simulink model "autoCreatedModel"  (R2023a)
settings: Solver=FixedStepDiscrete  StartTime=0.0  StopTime=10.0  FixedStep=0.1  RelTol=1e-3
undefined symbols (not defined in the file or in its folder): Batt_AncOutVoltage, Batt_BalancingRequired, Batt_BMSStatus, Batt_BoostChargeActive, Batt_ChargeContactorStatus, Batt_ClearFault_Code, Batt_ClearFault_KeyMatched, Batt_Coolant_IN_Pressure, Batt_Coolant_IN_Temp, Batt_Coolant_OUT_Pressure, Batt_Coolant_OUT_Temp, Batt_Current, Batt_DischargePowerLim, Batt_DischargePowerLim_2s, Batt_DischargePowerLim_5s, Batt_DischEnergyThroughput, Batt_EnergyAvailable, Batt_Equity_SoC_Displayed, Batt_Fault_FR0, Batt_Fault_FR1, Batt_Fault_FR2, Batt_Fault_FR3, Batt_Fault_FR4, Batt_Fault_FR5, Batt_Fault_FR6, Batt_Fault_FR7, Batt_FaultActive_FR4, Batt_HVILFault, Batt_InvOutVoltage, Batt_Isolation1OnOffStatus, Batt_Isolation1Res_HighRange, Batt_Isolation1Resistance, Batt_Isolation1Status, Batt_Isolation2OnOffStatus, Batt_Isolation2Status, Batt_LoggerPercent, Batt_LVBackupBattVoltage, Batt_LVVoltage, Batt_MainContactorStatus, Batt_MaxCellTemperature, Batt_MaxCellVoltage, Batt_MaxSOC, Batt_MinCellTemperature, Batt_MinCellVoltage, Batt_MinSOC, Batt_ReadyforBoostCharge, Batt_ReadytoTurnOnHV, Batt_RegenPowerLim, Batt_RegenPowerLim_2s, Batt_RegenPowerLim_5s, Batt_SafetyLightStatGreenHV, Batt_SafetyLightStatRedHV, Batt_SerialNumber, Batt_ThermalRequest, Batt_UserSOC, Batt_Voltage, BMS, BMS_AliveCounter1, BMS_AliveCounter2, BMS_AliveCounter3 ... (+154)
libraries: canoelib x133
(part 2 of 2)

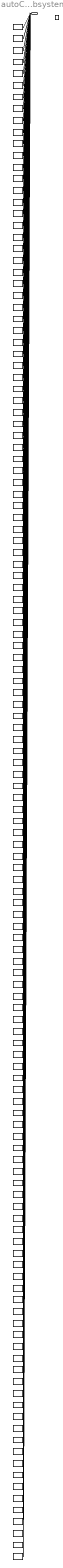
== system autoCreatedModel/BMS_EnabledSubsystem ==
  Enable : EnablePort
  En_OverRide_BMS_AliveCounter1 : canoelib/CANoe I//O/System Variable Input  nsName=HIL_Interface  sysVarName=CAN_OverRide::BMS::xC9_BMS_HV_01_Status::BMS_AliveCounter1::En_OverRide_BMS_AliveCounter1  arrayIndex=-1  editSampleTime=0.001  rawValue=Default  dataType=Default  dataTypeDB=unknown  hasEncoding=off  dataTypeCANoe=Get from CANoe
      settings: AttributesFormatString=%<nsName>::%<sysVarName>  SourceProductName=Vector CANoe
  En_OverRide_BMS_AliveCounter2 : canoelib/CANoe I//O/System Variable Input  nsName=HIL_Interface  sysVarName=CAN_OverRide::BMS::xCA_BMS_HV_02_HVParameter::BMS_AliveCounter2::En_OverRide_BMS_AliveCounter2  arrayIndex=-1  editSampleTime=0.001  rawValue=Default  dataType=Default  dataTypeDB=unknown  hasEncoding=off  dataTypeCANoe=Get from CANoe
      settings: AttributesFormatString=%<nsName>::%<sysVarName>  SourceProductName=Vector CANoe
  En_OverRide_BMS_AliveCounter3 : canoelib/CANoe I//O/System Variable Input  nsName=HIL_Interface  sysVarName=CAN_OverRide::BMS::xCB_BMS_HV_03_BatteryLimits::BMS_AliveCounter3::En_OverRide_BMS_AliveCounter3  arrayIndex=-1  editSampleTime=0.001  rawValue=Default  dataType=Default  dataTypeDB=unknown  hasEncoding=off  dataTypeCANoe=Get from CANoe
      settings: AttributesFormatString=%<nsName>::%<sysVarName>  SourceProductName=Vector CANoe
  En_OverRide_BMS_Calibration_info : canoelib/CANoe I//O/System Variable Input  nsName=HIL_Interface  sysVarName=CAN_OverRide::BMS::x112_BMS_HV_12::BMS_Calibration_info::En_OverRide_BMS_Calibration_info  arrayIndex=-1  editSampleTime=0.001  rawValue=Default  dataType=Default  dataTypeDB=unknown  hasEncoding=off  dataTypeCANoe=Get from CANoe
      settings: AttributesFormatString=%<nsName>::%<sysVarName>  SourceProductName=Vector CANoe
  En_OverRide_BMS_LoggingFull : canoelib/CANoe I//O/System Variable Input  nsName=HIL_Interface  sysVarName=CAN_OverRide::BMS::x110_BMS_HV_09::BMS_LoggingFull::En_OverRide_BMS_LoggingFull  arrayIndex=-1  editSampleTime=0.001  rawValue=Default  dataType=Default  dataTypeDB=unknown  hasEncoding=off  dataTypeCANoe=Get from CANoe
      settings: AttributesFormatString=%<nsName>::%<sysVarName>  SourceProductName=Vector CANoe
  En_OverRide_BMS_Software_info : canoelib/CANoe I//O/System Variable Input  nsName=HIL_Interface  sysVarName=CAN_OverRide::BMS::x112_BMS_HV_12::BMS_Software_info::En_OverRide_BMS_Software_info  arrayIndex=-1  editSampleTime=0.001  rawValue=Default  dataType=Default  dataTypeDB=unknown  hasEncoding=off  dataTypeCANoe=Get from CANoe
      settings: AttributesFormatString=%<nsName>::%<sysVarName>  SourceProductName=Vector CANoe
  En_OverRide_Batt_AncOutVoltage : canoelib/CANoe I//O/System Variable Input  nsName=HIL_Interface  sysVarName=CAN_OverRide::BMS::xCC_BMS_HV_04_ContactorStatus::Batt_AncOutVoltage::En_OverRide_Batt_AncOutVoltage  arrayIndex=-1  editSampleTime=0.001  rawValue=Default  dataType=Default  dataTypeDB=unknown  hasEncoding=off  dataTypeCANoe=Get from CANoe
      settings: AttributesFormatString=%<nsName>::%<sysVarName>  SourceProductName=Vector CANoe
  En_OverRide_Batt_BMSStatus : canoelib/CANoe I//O/System Variable Input  nsName=HIL_Interface  sysVarName=CAN_OverRide::BMS::xC9_BMS_HV_01_Status::Batt_BMSStatus::En_OverRide_Batt_BMSStatus  arrayIndex=-1  editSampleTime=0.001  rawValue=Default  dataType=Default  dataTypeDB=unknown  hasEncoding=off  dataTypeCANoe=Get from CANoe
      settings: AttributesFormatString=%<nsName>::%<sysVarName>  SourceProductName=Vector CANoe
  En_OverRide_Batt_BalancingRequired : canoelib/CANoe I//O/System Variable Input  nsName=HIL_Interface  sysVarName=CAN_OverRide::BMS::xC9_BMS_HV_01_Status::Batt_BalancingRequired::En_OverRide_Batt_BalancingRequired  arrayIndex=-1  editSampleTime=0.001  rawValue=Default  dataType=Default  dataTypeDB=unknown  hasEncoding=off  dataTypeCANoe=Get from CANoe
      settings: AttributesFormatString=%<nsName>::%<sysVarName>  SourceProductName=Vector CANoe
  En_OverRide_Batt_BoostChargeActive : canoelib/CANoe I//O/System Variable Input  nsName=HIL_Interface  sysVarName=CAN_OverRide::BMS::xD2_BMS_HV_08::Batt_BoostChargeActive::En_OverRide_Batt_BoostChargeActive  arrayIndex=-1  editSampleTime=0.001  rawValue=Default  dataType=Default  dataTypeDB=unknown  hasEncoding=off  dataTypeCANoe=Get from CANoe
      settings: AttributesFormatString=%<nsName>::%<sysVarName>  SourceProductName=Vector CANoe
  En_OverRide_Batt_ChargeContactorStatus : canoelib/CANoe I//O/System Variable Input  nsName=HIL_Interface  sysVarName=CAN_OverRide::BMS::xCC_BMS_HV_04_ContactorStatus::Batt_ChargeContactorStatus::En_OverRide_Batt_ChargeContactorStatus  arrayIndex=-1  editSampleTime=0.001  rawValue=Default  dataType=Default  dataTypeDB=unknown  hasEncoding=off  dataTypeCANoe=Get from CANoe
      settings: AttributesFormatString=%<nsName>::%<sysVarName>  SourceProductName=Vector CANoe
  En_OverRide_Batt_ClearFault_Code : canoelib/CANoe I//O/System Variable Input  nsName=HIL_Interface  sysVarName=CAN_OverRide::BMS::x110_BMS_HV_09::Batt_ClearFault_Code::En_OverRide_Batt_ClearFault_Code  arrayIndex=-1  editSampleTime=0.001  rawValue=Default  dataType=Default  dataTypeDB=unknown  hasEncoding=off  dataTypeCANoe=Get from CANoe
      settings: AttributesFormatString=%<nsName>::%<sysVarName>  SourceProductName=Vector CANoe
  En_OverRide_Batt_ClearFault_KeyMatched : canoelib/CANoe I//O/System Variable Input  nsName=HIL_Interface  sysVarName=CAN_OverRide::BMS::x110_BMS_HV_09::Batt_ClearFault_KeyMatched::En_OverRide_Batt_ClearFault_KeyMatched  arrayIndex=-1  editSampleTime=0.001  rawValue=Default  dataType=Default  dataTypeDB=unknown  hasEncoding=off  dataTypeCANoe=Get from CANoe
      settings: AttributesFormatString=%<nsName>::%<sysVarName>  SourceProductName=Vector CANoe
  En_OverRide_Batt_Coolant_IN_Pressure : canoelib/CANoe I//O/System Variable Input  nsName=HIL_Interface  sysVarName=CAN_OverRide::BMS::xCF_BMS_HV_07_Thermal::Batt_Coolant_IN_Pressure::En_OverRide_Batt_Coolant_IN_Pressure  arrayIndex=-1  editSampleTime=0.001  rawValue=Default  dataType=Default  dataTypeDB=unknown  hasEncoding=off  dataTypeCANoe=Get from CANoe
      settings: AttributesFormatString=%<nsName>::%<sysVarName>  SourceProductName=Vector CANoe
  En_OverRide_Batt_Coolant_IN_Temp : canoelib/CANoe I//O/System Variable Input  nsName=HIL_Interface  sysVarName=CAN_OverRide::BMS::xCF_BMS_HV_07_Thermal::Batt_Coolant_IN_Temp::En_OverRide_Batt_Coolant_IN_Temp  arrayIndex=-1  editSampleTime=0.001  rawValue=Default  dataType=Default  dataTypeDB=unknown  hasEncoding=off  dataTypeCANoe=Get from CANoe
      settings: AttributesFormatString=%<nsName>::%<sysVarName>  SourceProductName=Vector CANoe
  En_OverRide_Batt_Coolant_OUT_Pressure : canoelib/CANoe I//O/System Variable Input  nsName=HIL_Interface  sysVarName=CAN_OverRide::BMS::xCF_BMS_HV_07_Thermal::Batt_Coolant_OUT_Pressure::En_OverRide_Batt_Coolant_OUT_Pressure  arrayIndex=-1  editSampleTime=0.001  rawValue=Default  dataType=Default  dataTypeDB=unknown  hasEncoding=off  dataTypeCANoe=Get from CANoe
      settings: AttributesFormatString=%<nsName>::%<sysVarName>  SourceProductName=Vector CANoe
  En_OverRide_Batt_Coolant_OUT_Temp : canoelib/CANoe I//O/System Variable Input  nsName=HIL_Interface  sysVarName=CAN_OverRide::BMS::xCF_BMS_HV_07_Thermal::Batt_Coolant_OUT_Temp::En_OverRide_Batt_Coolant_OUT_Temp  arrayIndex=-1  editSampleTime=0.001  rawValue=Default  dataType=Default  dataTypeDB=unknown  hasEncoding=off  dataTypeCANoe=Get from CANoe
      settings: AttributesFormatString=%<nsName>::%<sysVarName>  SourceProductName=Vector CANoe
  En_OverRide_Batt_Current : canoelib/CANoe I//O/System Variable Input  nsName=HIL_Interface  sysVarName=CAN_OverRide::BMS::xCA_BMS_HV_02_HVParameter::Batt_Current::En_OverRide_Batt_Current  arrayIndex=-1  editSampleTime=0.001  rawValue=Default  dataType=Default  dataTypeDB=unknown  hasEncoding=off  dataTypeCANoe=Get from CANoe
      settings: AttributesFormatString=%<nsName>::%<sysVarName>  SourceProductName=Vector CANoe
  En_OverRide_Batt_DischEnergyThroughput : canoelib/CANoe I//O/System Variable Input  nsName=HIL_Interface  sysVarName=CAN_OverRide::BMS::xD2_BMS_HV_08::Batt_DischEnergyThroughput::En_OverRide_Batt_DischEnergyThroughput  arrayIndex=-1  editSampleTime=0.001  rawValue=Default  dataType=Default  dataTypeDB=unknown  hasEncoding=off  dataTypeCANoe=Get from CANoe
      settings: AttributesFormatString=%<nsName>::%<sysVarName>  SourceProductName=Vector CANoe
  En_OverRide_Batt_DischargePowerLim : canoelib/CANoe I//O/System Variable Input  nsName=HIL_Interface  sysVarName=CAN_OverRide::BMS::xCB_BMS_HV_03_BatteryLimits::Batt_DischargePowerLim::En_OverRide_Batt_DischargePowerLim  arrayIndex=-1  editSampleTime=0.001  rawValue=Default  dataType=Default  dataTypeDB=unknown  hasEncoding=off  dataTypeCANoe=Get from CANoe
      settings: AttributesFormatString=%<nsName>::%<sysVarName>  SourceProductName=Vector CANoe
  En_OverRide_Batt_DischargePowerLim_2s : canoelib/CANoe I//O/System Variable Input  nsName=HIL_Interface  sysVarName=CAN_OverRide::BMS::x109_BMS_HV_10::Batt_DischargePowerLim_2s::En_OverRide_Batt_DischargePowerLim_2s  arrayIndex=-1  editSampleTime=0.001  rawValue=Default  dataType=Default  dataTypeDB=unknown  hasEncoding=off  dataTypeCANoe=Get from CANoe
      settings: AttributesFormatString=%<nsName>::%<sysVarName>  SourceProductName=Vector CANoe
  En_OverRide_Batt_DischargePowerLim_5s : canoelib/CANoe I//O/System Variable Input  nsName=HIL_Interface  sysVarName=CAN_OverRide::BMS::x109_BMS_HV_10::Batt_DischargePowerLim_5s::En_OverRide_Batt_DischargePowerLim_5s  arrayIndex=-1  editSampleTime=0.001  rawValue=Default  dataType=Default  dataTypeDB=unknown  hasEncoding=off  dataTypeCANoe=Get from CANoe
      settings: AttributesFormatString=%<nsName>::%<sysVarName>  SourceProductName=Vector CANoe
  En_OverRide_Batt_EnergyAvailable : canoelib/CANoe I//O/System Variable Input  nsName=HIL_Interface  sysVarName=CAN_OverRide::BMS::xCE_BMS_HV_06::Batt_EnergyAvailable::En_OverRide_Batt_EnergyAvailable  arrayIndex=-1  editSampleTime=0.001  rawValue=Default  dataType=Default  dataTypeDB=unknown  hasEncoding=off  dataTypeCANoe=Get from CANoe
      settings: AttributesFormatString=%<nsName>::%<sysVarName>  SourceProductName=Vector CANoe
  En_OverRide_Batt_Equity_SoC_Displayed : canoelib/CANoe I//O/System Variable Input  nsName=HIL_Interface  sysVarName=CAN_OverRide::BMS::xC9_BMS_HV_01_Status::Batt_Equity_SoC_Displayed::En_OverRide_Batt_Equity_SoC_Displayed  arrayIndex=-1  editSampleTime=0.001  rawValue=Default  dataType=Default  dataTypeDB=unknown  hasEncoding=off  dataTypeCANoe=Get from CANoe
      settings: AttributesFormatString=%<nsName>::%<sysVarName>  SourceProductName=Vector CANoe
  En_OverRide_Batt_FaultActive_FR4 : canoelib/CANoe I//O/System Variable Input  nsName=HIL_Interface  sysVarName=CAN_OverRide::BMS::x110_BMS_HV_09::Batt_FaultActive_FR4::En_OverRide_Batt_FaultActive_FR4  arrayIndex=-1  editSampleTime=0.001  rawValue=Default  dataType=Default  dataTypeDB=unknown  hasEncoding=off  dataTypeCANoe=Get from CANoe
      settings: AttributesFormatString=%<nsName>::%<sysVarName>  SourceProductName=Vector CANoe
  En_OverRide_Batt_Fault_FR0 : canoelib/CANoe I//O/System Variable Input  nsName=HIL_Interface  sysVarName=CAN_OverRide::BMS::xC9_BMS_HV_01_Status::Batt_Fault_FR0::En_OverRide_Batt_Fault_FR0  arrayIndex=-1  editSampleTime=0.001  rawValue=Default  dataType=Default  dataTypeDB=unknown  hasEncoding=off  dataTypeCANoe=Get from CANoe
      settings: AttributesFormatString=%<nsName>::%<sysVarName>  SourceProductName=Vector CANoe
  En_OverRide_Batt_Fault_FR1 : canoelib/CANoe I//O/System Variable Input  nsName=HIL_Interface  sysVarName=CAN_OverRide::BMS::xC9_BMS_HV_01_Status::Batt_Fault_FR1::En_OverRide_Batt_Fault_FR1  arrayIndex=-1  editSampleTime=0.001  rawValue=Default  dataType=Default  dataTypeDB=unknown  hasEncoding=off  dataTypeCANoe=Get from CANoe
      settings: AttributesFormatString=%<nsName>::%<sysVarName>  SourceProductName=Vector CANoe
  En_OverRide_Batt_Fault_FR2 : canoelib/CANoe I//O/System Variable Input  nsName=HIL_Interface  sysVarName=CAN_OverRide::BMS::xC9_BMS_HV_01_Status::Batt_Fault_FR2::En_OverRide_Batt_Fault_FR2  arrayIndex=-1  editSampleTime=0.001  rawValue=Default  dataType=Default  dataTypeDB=unknown  hasEncoding=off  dataTypeCANoe=Get from CANoe
      settings: AttributesFormatString=%<nsName>::%<sysVarName>  SourceProductName=Vector CANoe
  En_OverRide_Batt_Fault_FR3 : canoelib/CANoe I//O/System Variable Input  nsName=HIL_Interface  sysVarName=CAN_OverRide::BMS::xC9_BMS_HV_01_Status::Batt_Fault_FR3::En_OverRide_Batt_Fault_FR3  arrayIndex=-1  editSampleTime=0.001  rawValue=Default  dataType=Default  dataTypeDB=unknown  hasEncoding=off  dataTypeCANoe=Get from CANoe
      settings: AttributesFormatString=%<nsName>::%<sysVarName>  SourceProductName=Vector CANoe
  En_OverRide_Batt_Fault_FR4 : canoelib/CANoe I//O/System Variable Input  nsName=HIL_Interface  sysVarName=CAN_OverRide::BMS::xC9_BMS_HV_01_Status::Batt_Fault_FR4::En_OverRide_Batt_Fault_FR4  arrayIndex=-1  editSampleTime=0.001  rawValue=Default  dataType=Default  dataTypeDB=unknown  hasEncoding=off  dataTypeCANoe=Get from CANoe
      settings: AttributesFormatString=%<nsName>::%<sysVarName>  SourceProductName=Vector CANoe
  En_OverRide_Batt_Fault_FR5 : canoelib/CANoe I//O/System Variable Input  nsName=HIL_Interface  sysVarName=CAN_OverRide::BMS::xC9_BMS_HV_01_Status::Batt_Fault_FR5::En_OverRide_Batt_Fault_FR5  arrayIndex=-1  editSampleTime=0.001  rawValue=Default  dataType=Default  dataTypeDB=unknown  hasEncoding=off  dataTypeCANoe=Get from CANoe
      settings: AttributesFormatString=%<nsName>::%<sysVarName>  SourceProductName=Vector CANoe
  En_OverRide_Batt_Fault_FR6 : canoelib/CANoe I//O/System Variable Input  nsName=HIL_Interface  sysVarName=CAN_OverRide::BMS::xC9_BMS_HV_01_Status::Batt_Fault_FR6::En_OverRide_Batt_Fault_FR6  arrayIndex=-1  editSampleTime=0.001  rawValue=Default  dataType=Default  dataTypeDB=unknown  hasEncoding=off  dataTypeCANoe=Get from CANoe
      settings: AttributesFormatString=%<nsName>::%<sysVarName>  SourceProductName=Vector CANoe
  En_OverRide_Batt_Fault_FR7 : canoelib/CANoe I//O/System Variable Input  nsName=HIL_Interface  sysVarName=CAN_OverRide::BMS::xC9_BMS_HV_01_Status::Batt_Fault_FR7::En_OverRide_Batt_Fault_FR7  arrayIndex=-1  editSampleTime=0.001  rawValue=Default  dataType=Default  dataTypeDB=unknown  hasEncoding=off  dataTypeCANoe=Get from CANoe
      settings: AttributesFormatString=%<nsName>::%<sysVarName>  SourceProductName=Vector CANoe
  En_OverRide_Batt_HVILFault : canoelib/CANoe I//O/System Variable Input  nsName=HIL_Interface  sysVarName=CAN_OverRide::BMS::xC9_BMS_HV_01_Status::Batt_HVILFault::En_OverRide_Batt_HVILFault  arrayIndex=-1  editSampleTime=0.001  rawValue=Default  dataType=Default  dataTypeDB=unknown  hasEncoding=off  dataTypeCANoe=Get from CANoe
      settings: AttributesFormatString=%<nsName>::%<sysVarName>  SourceProductName=Vector CANoe
  En_OverRide_Batt_InvOutVoltage : canoelib/CANoe I//O/System Variable Input  nsName=HIL_Interface  sysVarName=CAN_OverRide::BMS::xCC_BMS_HV_04_ContactorStatus::Batt_InvOutVoltage::En_OverRide_Batt_InvOutVoltage  arrayIndex=-1  editSampleTime=0.001  rawValue=Default  dataType=Default  dataTypeDB=unknown  hasEncoding=off  dataTypeCANoe=Get from CANoe
      settings: AttributesFormatString=%<nsName>::%<sysVarName>  SourceProductName=Vector CANoe
  En_OverRide_Batt_Isolation1OnOffStatus : canoelib/CANoe I//O/System Variable Input  nsName=HIL_Interface  sysVarName=CAN_OverRide::BMS::xC9_BMS_HV_01_Status::Batt_Isolation1OnOffStatus::En_OverRide_Batt_Isolation1OnOffStatus  arrayIndex=-1  editSampleTime=0.001  rawValue=Default  dataType=Default  dataTypeDB=unknown  hasEncoding=off  dataTypeCANoe=Get from CANoe
      settings: AttributesFormatString=%<nsName>::%<sysVarName>  SourceProductName=Vector CANoe
  En_OverRide_Batt_Isolation1Res_HighRange : canoelib/CANoe I//O/System Variable Input  nsName=HIL_Interface  sysVarName=CAN_OverRide::BMS::xCE_BMS_HV_06::Batt_Isolation1Res_HighRange::En_OverRide_Batt_Isolation1Res_HighRange  arrayIndex=-1  editSampleTime=0.001  rawValue=Default  dataType=Default  dataTypeDB=unknown  hasEncoding=off  dataTypeCANoe=Get from CANoe
      settings: AttributesFormatString=%<nsName>::%<sysVarName>  SourceProductName=Vector CANoe
  En_OverRide_Batt_Isolation1Resistance : canoelib/CANoe I//O/System Variable Input  nsName=HIL_Interface  sysVarName=CAN_OverRide::BMS::xCE_BMS_HV_06::Batt_Isolation1Resistance::En_OverRide_Batt_Isolation1Resistance  arrayIndex=-1  editSampleTime=0.001  rawValue=Default  dataType=Default  dataTypeDB=unknown  hasEncoding=off  dataTypeCANoe=Get from CANoe
      settings: AttributesFormatString=%<nsName>::%<sysVarName>  SourceProductName=Vector CANoe
  En_OverRide_Batt_Isolation1Status : canoelib/CANoe I//O/System Variable Input  nsName=HIL_Interface  sysVarName=CAN_OverRide::BMS::xC9_BMS_HV_01_Status::Batt_Isolation1Status::En_OverRide_Batt_Isolation1Status  arrayIndex=-1  editSampleTime=0.001  rawValue=Default  dataType=Default  dataTypeDB=unknown  hasEncoding=off  dataTypeCANoe=Get from CANoe
      settings: AttributesFormatString=%<nsName>::%<sysVarName>  SourceProductName=Vector CANoe
  En_OverRide_Batt_Isolation2OnOffStatus : canoelib/CANoe I//O/System Variable Input  nsName=HIL_Interface  sysVarName=CAN_OverRide::BMS::xC9_BMS_HV_01_Status::Batt_Isolation2OnOffStatus::En_OverRide_Batt_Isolation2OnOffStatus  arrayIndex=-1  editSampleTime=0.001  rawValue=Default  dataType=Default  dataTypeDB=unknown  hasEncoding=off  dataTypeCANoe=Get from CANoe
      settings: AttributesFormatString=%<nsName>::%<sysVarName>  SourceProductName=Vector CANoe
  En_OverRide_Batt_Isolation2Status : canoelib/CANoe I//O/System Variable Input  nsName=HIL_Interface  sysVarName=CAN_OverRide::BMS::xC9_BMS_HV_01_Status::Batt_Isolation2Status::En_OverRide_Batt_Isolation2Status  arrayIndex=-1  editSampleTime=0.001  rawValue=Default  dataType=Default  dataTypeDB=unknown  hasEncoding=off  dataTypeCANoe=Get from CANoe
      settings: AttributesFormatString=%<nsName>::%<sysVarName>  SourceProductName=Vector CANoe
  En_OverRide_Batt_LVBackupBattVoltage : canoelib/CANoe I//O/System Variable Input  nsName=HIL_Interface  sysVarName=CAN_OverRide::BMS::xCF_BMS_HV_07_Thermal::Batt_LVBackupBattVoltage::En_OverRide_Batt_LVBackupBattVoltage  arrayIndex=-1  editSampleTime=0.001  rawValue=Default  dataType=Default  dataTypeDB=unknown  hasEncoding=off  dataTypeCANoe=Get from CANoe
      settings: AttributesFormatString=%<nsName>::%<sysVarName>  SourceProductName=Vector CANoe
  En_OverRide_Batt_LVVoltage : canoelib/CANoe I//O/System Variable Input  nsName=HIL_Interface  sysVarName=CAN_OverRide::BMS::xCE_BMS_HV_06::Batt_LVVoltage::En_OverRide_Batt_LVVoltage  arrayIndex=-1  editSampleTime=0.001  rawValue=Default  dataType=Default  dataTypeDB=unknown  hasEncoding=off  dataTypeCANoe=Get from CANoe
      settings: AttributesFormatString=%<nsName>::%<sysVarName>  SourceProductName=Vector CANoe
  En_OverRide_Batt_LoggerPercent : canoelib/CANoe I//O/System Variable Input  nsName=HIL_Interface  sysVarName=CAN_OverRide::BMS::x110_BMS_HV_09::Batt_LoggerPercent::En_OverRide_Batt_LoggerPercent  arrayIndex=-1  editSampleTime=0.001  rawValue=Default  dataType=Default  dataTypeDB=unknown  hasEncoding=off  dataTypeCANoe=Get from CANoe
      settings: AttributesFormatString=%<nsName>::%<sysVarName>  SourceProductName=Vector CANoe
  En_OverRide_Batt_MainContactorStatus : canoelib/CANoe I//O/System Variable Input  nsName=HIL_Interface  sysVarName=CAN_OverRide::BMS::xCC_BMS_HV_04_ContactorStatus::Batt_MainContactorStatus::En_OverRide_Batt_MainContactorStatus  arrayIndex=-1  editSampleTime=0.001  rawValue=Default  dataType=Default  dataTypeDB=unknown  hasEncoding=off  dataTypeCANoe=Get from CANoe
      settings: AttributesFormatString=%<nsName>::%<sysVarName>  SourceProductName=Vector CANoe
  En_OverRide_Batt_MaxCellTemperature : canoelib/CANoe I//O/System Variable Input  nsName=HIL_Interface  sysVarName=CAN_OverRide::BMS::xCD_BMS_HV_05_CellParam::Batt_MaxCellTemperature::En_OverRide_Batt_MaxCellTemperature  arrayIndex=-1  editSampleTime=0.001  rawValue=Default  dataType=Default  dataTypeDB=unknown  hasEncoding=off  dataTypeCANoe=Get from CANoe
      settings: AttributesFormatString=%<nsName>::%<sysVarName>  SourceProductName=Vector CANoe
  En_OverRide_Batt_MaxCellVoltage : canoelib/CANoe I//O/System Variable Input  nsName=HIL_Interface  sysVarName=CAN_OverRide::BMS::xCD_BMS_HV_05_CellParam::Batt_MaxCellVoltage::En_OverRide_Batt_MaxCellVoltage  arrayIndex=-1  editSampleTime=0.001  rawValue=Default  dataType=Default  dataTypeDB=unknown  hasEncoding=off  dataTypeCANoe=Get from CANoe
      settings: AttributesFormatString=%<nsName>::%<sysVarName>  SourceProductName=Vector CANoe
  En_OverRide_Batt_MaxSOC : canoelib/CANoe I//O/System Variable Input  nsName=HIL_Interface  sysVarName=CAN_OverRide::BMS::x110_BMS_HV_09::Batt_MaxSOC::En_OverRide_Batt_MaxSOC  arrayIndex=-1  editSampleTime=0.001  rawValue=Default  dataType=Default  dataTypeDB=unknown  hasEncoding=off  dataTypeCANoe=Get from CANoe
      settings: AttributesFormatString=%<nsName>::%<sysVarName>  SourceProductName=Vector CANoe
  En_OverRide_Batt_MinCellTemperature : canoelib/CANoe I//O/System Variable Input  nsName=HIL_Interface  sysVarName=CAN_OverRide::BMS::xCD_BMS_HV_05_CellParam::Batt_MinCellTemperature::En_OverRide_Batt_MinCellTemperature  arrayIndex=-1  editSampleTime=0.001  rawValue=Default  dataType=Default  dataTypeDB=unknown  hasEncoding=off  dataTypeCANoe=Get from CANoe
      settings: AttributesFormatString=%<nsName>::%<sysVarName>  SourceProductName=Vector CANoe
  En_OverRide_Batt_MinCellVoltage : canoelib/CANoe I//O/System Variable Input  nsName=HIL_Interface  sysVarName=CAN_OverRide::BMS::xCD_BMS_HV_05_CellParam::Batt_MinCellVoltage::En_OverRide_Batt_MinCellVoltage  arrayIndex=-1  editSampleTime=0.001  rawValue=Default  dataType=Default  dataTypeDB=unknown  hasEncoding=off  dataTypeCANoe=Get from CANoe
      settings: AttributesFormatString=%<nsName>::%<sysVarName>  SourceProductName=Vector CANoe
  En_OverRide_Batt_MinSOC : canoelib/CANoe I//O/System Variable Input  nsName=HIL_Interface  sysVarName=CAN_OverRide::BMS::xC9_BMS_HV_01_Status::Batt_MinSOC::En_OverRide_Batt_MinSOC  arrayIndex=-1  editSampleTime=0.001  rawValue=Default  dataType=Default  dataTypeDB=unknown  hasEncoding=off  dataTypeCANoe=Get from CANoe
      settings: AttributesFormatString=%<nsName>::%<sysVarName>  SourceProductName=Vector CANoe
  En_OverRide_Batt_ReadyforBoostCharge : canoelib/CANoe I//O/System Variable Input  nsName=HIL_Interface  sysVarName=CAN_OverRide::BMS::xD2_BMS_HV_08::Batt_ReadyforBoostCharge::En_OverRide_Batt_ReadyforBoostCharge  arrayIndex=-1  editSampleTime=0.001  rawValue=Default  dataType=Default  dataTypeDB=unknown  hasEncoding=off  dataTypeCANoe=Get from CANoe
      settings: AttributesFormatString=%<nsName>::%<sysVarName>  SourceProductName=Vector CANoe
  En_OverRide_Batt_ReadytoTurnOnHV : canoelib/CANoe I//O/System Variable Input  nsName=HIL_Interface  sysVarName=CAN_OverRide::BMS::xC9_BMS_HV_01_Status::Batt_ReadytoTurnOnHV::En_OverRide_Batt_ReadytoTurnOnHV  arrayIndex=-1  editSampleTime=0.001  rawValue=Default  dataType=Default  dataTypeDB=unknown  hasEncoding=off  dataTypeCANoe=Get from CANoe
      settings: AttributesFormatString=%<nsName>::%<sysVarName>  SourceProductName=Vector CANoe
  En_OverRide_Batt_RegenPowerLim : canoelib/CANoe I//O/System Variable Input  nsName=HIL_Interface  sysVarName=CAN_OverRide::BMS::xCB_BMS_HV_03_BatteryLimits::Batt_RegenPowerLim::En_OverRide_Batt_RegenPowerLim  arrayIndex=-1  editSampleTime=0.001  rawValue=Default  dataType=Default  dataTypeDB=unknown  hasEncoding=off  dataTypeCANoe=Get from CANoe
      settings: AttributesFormatString=%<nsName>::%<sysVarName>  SourceProductName=Vector CANoe
  En_OverRide_Batt_RegenPowerLim_2s : canoelib/CANoe I//O/System Variable Input  nsName=HIL_Interface  sysVarName=CAN_OverRide::BMS::x109_BMS_HV_10::Batt_RegenPowerLim_2s::En_OverRide_Batt_RegenPowerLim_2s  arrayIndex=-1  editSampleTime=0.001  rawValue=Default  dataType=Default  dataTypeDB=unknown  hasEncoding=off  dataTypeCANoe=Get from CANoe
      settings: AttributesFormatString=%<nsName>::%<sysVarName>  SourceProductName=Vector CANoe
  En_OverRide_Batt_RegenPowerLim_5s : canoelib/CANoe I//O/System Variable Input  nsName=HIL_Interface  sysVarName=CAN_OverRide::BMS::x109_BMS_HV_10::Batt_RegenPowerLim_5s::En_OverRide_Batt_RegenPowerLim_5s  arrayIndex=-1  editSampleTime=0.001  rawValue=Default  dataType=Default  dataTypeDB=unknown  hasEncoding=off  dataTypeCANoe=Get from CANoe
      settings: AttributesFormatString=%<nsName>::%<sysVarName>  SourceProductName=Vector CANoe
  En_OverRide_Batt_SafetyLightStatGreenHV : canoelib/CANoe I//O/System Variable Input  nsName=HIL_Interface  sysVarName=CAN_OverRide::BMS::xD2_BMS_HV_08::Batt_SafetyLightStatGreenHV::En_OverRide_Batt_SafetyLightStatGreenHV  arrayIndex=-1  editSampleTime=0.001  rawValue=Default  dataType=Default  dataTypeDB=unknown  hasEncoding=off  dataTypeCANoe=Get from CANoe
      settings: AttributesFormatString=%<nsName>::%<sysVarName>  SourceProductName=Vector CANoe
  En_OverRide_Batt_SafetyLightStatRedHV : canoelib/CANoe I//O/System Variable Input  nsName=HIL_Interface  sysVarName=CAN_OverRide::BMS::xD2_BMS_HV_08::Batt_SafetyLightStatRedHV::En_OverRide_Batt_SafetyLightStatRedHV  arrayIndex=-1  editSampleTime=0.001  rawValue=Default  dataType=Default  dataTypeDB=unknown  hasEncoding=off  dataTypeCANoe=Get from CANoe
      settings: AttributesFormatString=%<nsName>::%<sysVarName>  SourceProductName=Vector CANoe
  En_OverRide_Batt_SerialNumber : canoelib/CANoe I//O/System Variable Input  nsName=HIL_Interface  sysVarName=CAN_OverRide::BMS::x112_BMS_HV_12::Batt_SerialNumber::En_OverRide_Batt_SerialNumber  arrayIndex=-1  editSampleTime=0.001  rawValue=Default  dataType=Default  dataTypeDB=unknown  hasEncoding=off  dataTypeCANoe=Get from CANoe
      settings: AttributesFormatString=%<nsName>::%<sysVarName>  SourceProductName=Vector CANoe
  En_OverRide_Batt_ThermalRequest : canoelib/CANoe I//O/System Variable Input  nsName=HIL_Interface  sysVarName=CAN_OverRide::BMS::xCF_BMS_HV_07_Thermal::Batt_ThermalRequest::En_OverRide_Batt_ThermalRequest  arrayIndex=-1  editSampleTime=0.001  rawValue=Default  dataType=Default  dataTypeDB=unknown  hasEncoding=off  dataTypeCANoe=Get from CANoe
      settings: AttributesFormatString=%<nsName>::%<sysVarName>  SourceProductName=Vector CANoe
  En_OverRide_Batt_UserSOC : canoelib/CANoe I//O/System Variable Input  nsName=HIL_Interface  sysVarName=CAN_OverRide::BMS::xC9_BMS_HV_01_Status::Batt_UserSOC::En_OverRide_Batt_UserSOC  arrayIndex=-1  editSampleTime=0.001  rawValue=Default  dataType=Default  dataTypeDB=unknown  hasEncoding=off  dataTypeCANoe=Get from CANoe
      settings: AttributesFormatString=%<nsName>::%<sysVarName>  SourceProductName=Vector CANoe
  En_OverRide_Batt_Voltage : canoelib/CANoe I//O/System Variable Input  nsName=HIL_Interface  sysVarName=CAN_OverRide::BMS::xCA_BMS_HV_02_HVParameter::Batt_Voltage::En_OverRide_Batt_Voltage  arrayIndex=-1  editSampleTime=0.001  rawValue=Default  dataType=Default  dataTypeDB=unknown  hasEncoding=off  dataTypeCANoe=Get from CANoe
      settings: AttributesFormatString=%<nsName>::%<sysVarName>  SourceProductName=Vector CANoe
  En_OverRide_CIM_ChargePlugLockStatusHV : canoelib/CANoe I//O/System Variable Input  nsName=HIL_Interface  sysVarName=CAN_OverRide::BMS::x12D_CIM_HV_01::CIM_ChargePlugLockStatusHV::En_OverRide_CIM_ChargePlugLockStatusHV  arrayIndex=-1  editSampleTime=0.001  rawValue=Default  dataType=Default  dataTypeDB=unknown  hasEncoding=off  dataTypeCANoe=Get from CANoe
      settings: AttributesFormatString=%<nsName>::%<sysVarName>  SourceProductName=Vector CANoe
  En_OverRide_CIM_ChargeStatusHV : canoelib/CANoe I//O/System Variable Input  nsName=HIL_Interface  sysVarName=CAN_OverRide::BMS::x12D_CIM_HV_01::CIM_ChargeStatusHV::En_OverRide_CIM_ChargeStatusHV  arrayIndex=-1  editSampleTime=0.001  rawValue=Default  dataType=Default  dataTypeDB=unknown  hasEncoding=off  dataTypeCANoe=Get from CANoe
      settings: AttributesFormatString=%<nsName>::%<sysVarName>  SourceProductName=Vector CANoe
  En_OverRide_CIM_ChargingPlugTypeHV : canoelib/CANoe I//O/System Variable Input  nsName=HIL_Interface  sysVarName=CAN_OverRide::BMS::x12D_CIM_HV_01::CIM_ChargingPlugTypeHV::En_OverRide_CIM_ChargingPlugTypeHV  arrayIndex=-1  editSampleTime=0.001  rawValue=Default  dataType=Default  dataTypeDB=unknown  hasEncoding=off  dataTypeCANoe=Get from CANoe
      settings: AttributesFormatString=%<nsName>::%<sysVarName>  SourceProductName=Vector CANoe
  En_OverRide_CIM_PlugPresentHV : canoelib/CANoe I//O/System Variable Input  nsName=HIL_Interface  sysVarName=CAN_OverRide::BMS::x12D_CIM_HV_01::CIM_PlugPresentHV::En_OverRide_CIM_PlugPresentHV  arrayIndex=-1  editSampleTime=0.001  rawValue=Default  dataType=Default  dataTypeDB=unknown  hasEncoding=off  dataTypeCANoe=Get from CANoe
      settings: AttributesFormatString=%<nsName>::%<sysVarName>  SourceProductName=Vector CANoe
  Val_OverRide_BMS_AliveCounter1 : canoelib/CANoe I//O/System Variable Input  nsName=HIL_Interface  sysVarName=CAN_OverRide::BMS::xC9_BMS_HV_01_Status::BMS_AliveCounter1::Val_OverRide_BMS_AliveCounter1  arrayIndex=-1  editSampleTime=0.001  rawValue=Default  dataType=Default  dataTypeDB=unknown  hasEncoding=off  dataTypeCANoe=Get from CANoe
      settings: AttributesFormatString=%<nsName>::%<sysVarName>  SourceProductName=Vector CANoe
  Val_OverRide_BMS_AliveCounter2 : canoelib/CANoe I//O/System Variable Input  nsName=HIL_Interface  sysVarName=CAN_OverRide::BMS::xCA_BMS_HV_02_HVParameter::BMS_AliveCounter2::Val_OverRide_BMS_AliveCounter2  arrayIndex=-1  editSampleTime=0.001  rawValue=Default  dataType=Default  dataTypeDB=unknown  hasEncoding=off  dataTypeCANoe=Get from CANoe
      settings: AttributesFormatString=%<nsName>::%<sysVarName>  SourceProductName=Vector CANoe
  Val_OverRide_BMS_AliveCounter3 : canoelib/CANoe I//O/System Variable Input  nsName=HIL_Interface  sysVarName=CAN_OverRide::BMS::xCB_BMS_HV_03_BatteryLimits::BMS_AliveCounter3::Val_OverRide_BMS_AliveCounter3  arrayIndex=-1  editSampleTime=0.001  rawValue=Default  dataType=Default  dataTypeDB=unknown  hasEncoding=off  dataTypeCANoe=Get from CANoe
      settings: AttributesFormatString=%<nsName>::%<sysVarName>  SourceProductName=Vector CANoe
  Val_OverRide_BMS_Calibration_info : canoelib/CANoe I//O/System Variable Input  nsName=HIL_Interface  sysVarName=CAN_OverRide::BMS::x112_BMS_HV_12::BMS_Calibration_info::Val_OverRide_BMS_Calibration_info  arrayIndex=-1  editSampleTime=0.001  rawValue=Default  dataType=Default  dataTypeDB=unknown  hasEncoding=off  dataTypeCANoe=Get from CANoe
      settings: AttributesFormatString=%<nsName>::%<sysVarName>  SourceProductName=Vector CANoe
  Val_OverRide_BMS_LoggingFull : canoelib/CANoe I//O/System Variable Input  nsName=HIL_Interface  sysVarName=CAN_OverRide::BMS::x110_BMS_HV_09::BMS_LoggingFull::Val_OverRide_BMS_LoggingFull  arrayIndex=-1  editSampleTime=0.001  rawValue=Default  dataType=Default  dataTypeDB=unknown  hasEncoding=off  dataTypeCANoe=Get from CANoe
      settings: AttributesFormatString=%<nsName>::%<sysVarName>  SourceProductName=Vector CANoe
  Val_OverRide_BMS_Software_info : canoelib/CANoe I//O/System Variable Input  nsName=HIL_Interface  sysVarName=CAN_OverRide::BMS::x112_BMS_HV_12::BMS_Software_info::Val_OverRide_BMS_Software_info  arrayIndex=-1  editSampleTime=0.001  rawValue=Default  dataType=Default  dataTypeDB=unknown  hasEncoding=off  dataTypeCANoe=Get from CANoe
      settings: AttributesFormatString=%<nsName>::%<sysVarName>  SourceProductName=Vector CANoe
  Val_OverRide_Batt_AncOutVoltage : canoelib/CANoe I//O/System Variable Input  nsName=HIL_Interface  sysVarName=CAN_OverRide::BMS::xCC_BMS_HV_04_ContactorStatus::Batt_AncOutVoltage::Val_OverRide_Batt_AncOutVoltage  arrayIndex=-1  editSampleTime=0.001  rawValue=Default  dataType=Default  dataTypeDB=unknown  hasEncoding=off  dataTypeCANoe=Get from CANoe
      settings: AttributesFormatString=%<nsName>::%<sysVarName>  SourceProductName=Vector CANoe
  Val_OverRide_Batt_BMSStatus : canoelib/CANoe I//O/System Variable Input  nsName=HIL_Interface  sysVarName=CAN_OverRide::BMS::xC9_BMS_HV_01_Status::Batt_BMSStatus::Val_OverRide_Batt_BMSStatus  arrayIndex=-1  editSampleTime=0.001  rawValue=Default  dataType=Default  dataTypeDB=unknown  hasEncoding=off  dataTypeCANoe=Get from CANoe
      settings: AttributesFormatString=%<nsName>::%<sysVarName>  SourceProductName=Vector CANoe
  Val_OverRide_Batt_BalancingRequired : canoelib/CANoe I//O/System Variable Input  nsName=HIL_Interface  sysVarName=CAN_OverRide::BMS::xC9_BMS_HV_01_Status::Batt_BalancingRequired::Val_OverRide_Batt_BalancingRequired  arrayIndex=-1  editSampleTime=0.001  rawValue=Default  dataType=Default  dataTypeDB=unknown  hasEncoding=off  dataTypeCANoe=Get from CANoe
      settings: AttributesFormatString=%<nsName>::%<sysVarName>  SourceProductName=Vector CANoe
  Val_OverRide_Batt_BoostChargeActive : canoelib/CANoe I//O/System Variable Input  nsName=HIL_Interface  sysVarName=CAN_OverRide::BMS::xD2_BMS_HV_08::Batt_BoostChargeActive::Val_OverRide_Batt_BoostChargeActive  arrayIndex=-1  editSampleTime=0.001  rawValue=Default  dataType=Default  dataTypeDB=unknown  hasEncoding=off  dataTypeCANoe=Get from CANoe
      settings: AttributesFormatString=%<nsName>::%<sysVarName>  SourceProductName=Vector CANoe
  Val_OverRide_Batt_ChargeContactorStatus : canoelib/CANoe I//O/System Variable Input  nsName=HIL_Interface  sysVarName=CAN_OverRide::BMS::xCC_BMS_HV_04_ContactorStatus::Batt_ChargeContactorStatus::Val_OverRide_Batt_ChargeContactorStatus  arrayIndex=-1  editSampleTime=0.001  rawValue=Default  dataType=Default  dataTypeDB=unknown  hasEncoding=off  dataTypeCANoe=Get from CANoe
      settings: AttributesFormatString=%<nsName>::%<sysVarName>  SourceProductName=Vector CANoe
  Val_OverRide_Batt_ClearFault_Code : canoelib/CANoe I//O/System Variable Input  nsName=HIL_Interface  sysVarName=CAN_OverRide::BMS::x110_BMS_HV_09::Batt_ClearFault_Code::Val_OverRide_Batt_ClearFault_Code  arrayIndex=-1  editSampleTime=0.001  rawValue=Default  dataType=Default  dataTypeDB=unknown  hasEncoding=off  dataTypeCANoe=Get from CANoe
      settings: AttributesFormatString=%<nsName>::%<sysVarName>  SourceProductName=Vector CANoe
  Val_OverRide_Batt_ClearFault_KeyMatched : canoelib/CANoe I//O/System Variable Input  nsName=HIL_Interface  sysVarName=CAN_OverRide::BMS::x110_BMS_HV_09::Batt_ClearFault_KeyMatched::Val_OverRide_Batt_ClearFault_KeyMatched  arrayIndex=-1  editSampleTime=0.001  rawValue=Default  dataType=Default  dataTypeDB=unknown  hasEncoding=off  dataTypeCANoe=Get from CANoe
      settings: AttributesFormatString=%<nsName>::%<sysVarName>  SourceProductName=Vector CANoe
  Val_OverRide_Batt_Coolant_IN_Pressure : canoelib/CANoe I//O/System Variable Input  nsName=HIL_Interface  sysVarName=CAN_OverRide::BMS::xCF_BMS_HV_07_Thermal::Batt_Coolant_IN_Pressure::Val_OverRide_Batt_Coolant_IN_Pressure  arrayIndex=-1  editSampleTime=0.001  rawValue=Default  dataType=Default  dataTypeDB=unknown  hasEncoding=off  dataTypeCANoe=Get from CANoe
      settings: AttributesFormatString=%<nsName>::%<sysVarName>  SourceProductName=Vector CANoe
  Val_OverRide_Batt_Coolant_IN_Temp : canoelib/CANoe I//O/System Variable Input  nsName=HIL_Interface  sysVarName=CAN_OverRide::BMS::xCF_BMS_HV_07_Thermal::Batt_Coolant_IN_Temp::Val_OverRide_Batt_Coolant_IN_Temp  arrayIndex=-1  editSampleTime=0.001  rawValue=Default  dataType=Default  dataTypeDB=unknown  hasEncoding=off  dataTypeCANoe=Get from CANoe
      settings: AttributesFormatString=%<nsName>::%<sysVarName>  SourceProductName=Vector CANoe
  Val_OverRide_Batt_Coolant_OUT_Pressure : canoelib/CANoe I//O/System Variable Input  nsName=HIL_Interface  sysVarName=CAN_OverRide::BMS::xCF_BMS_HV_07_Thermal::Batt_Coolant_OUT_Pressure::Val_OverRide_Batt_Coolant_OUT_Pressure  arrayIndex=-1  editSampleTime=0.001  rawValue=Default  dataType=Default  dataTypeDB=unknown  hasEncoding=off  dataTypeCANoe=Get from CANoe
      settings: AttributesFormatString=%<nsName>::%<sysVarName>  SourceProductName=Vector CANoe
  Val_OverRide_Batt_Coolant_OUT_Temp : canoelib/CANoe I//O/System Variable Input  nsName=HIL_Interface  sysVarName=CAN_OverRide::BMS::xCF_BMS_HV_07_Thermal::Batt_Coolant_OUT_Temp::Val_OverRide_Batt_Coolant_OUT_Temp  arrayIndex=-1  editSampleTime=0.001  rawValue=Default  dataType=Default  dataTypeDB=unknown  hasEncoding=off  dataTypeCANoe=Get from CANoe
      settings: AttributesFormatString=%<nsName>::%<sysVarName>  SourceProductName=Vector CANoe
  Val_OverRide_Batt_Current : canoelib/CANoe I//O/System Variable Input  nsName=HIL_Interface  sysVarName=CAN_OverRide::BMS::xCA_BMS_HV_02_HVParameter::Batt_Current::Val_OverRide_Batt_Current  arrayIndex=-1  editSampleTime=0.001  rawValue=Default  dataType=Default  dataTypeDB=unknown  hasEncoding=off  dataTypeCANoe=Get from CANoe
      settings: AttributesFormatString=%<nsName>::%<sysVarName>  SourceProductName=Vector CANoe
  Val_OverRide_Batt_DischEnergyThroughput : canoelib/CANoe I//O/System Variable Input  nsName=HIL_Interface  sysVarName=CAN_OverRide::BMS::xD2_BMS_HV_08::Batt_DischEnergyThroughput::Val_OverRide_Batt_DischEnergyThroughput  arrayIndex=-1  editSampleTime=0.001  rawValue=Default  dataType=Default  dataTypeDB=unknown  hasEncoding=off  dataTypeCANoe=Get from CANoe
      settings: AttributesFormatString=%<nsName>::%<sysVarName>  SourceProductName=Vector CANoe
  Val_OverRide_Batt_DischargePowerLim : canoelib/CANoe I//O/System Variable Input  nsName=HIL_Interface  sysVarName=CAN_OverRide::BMS::xCB_BMS_HV_03_BatteryLimits::Batt_DischargePowerLim::Val_OverRide_Batt_DischargePowerLim  arrayIndex=-1  editSampleTime=0.001  rawValue=Default  dataType=Default  dataTypeDB=unknown  hasEncoding=off  dataTypeCANoe=Get from CANoe
      settings: AttributesFormatString=%<nsName>::%<sysVarName>  SourceProductName=Vector CANoe
  Val_OverRide_Batt_DischargePowerLim_2s : canoelib/CANoe I//O/System Variable Input  nsName=HIL_Interface  sysVarName=CAN_OverRide::BMS::x109_BMS_HV_10::Batt_DischargePowerLim_2s::Val_OverRide_Batt_DischargePowerLim_2s  arrayIndex=-1  editSampleTime=0.001  rawValue=Default  dataType=Default  dataTypeDB=unknown  hasEncoding=off  dataTypeCANoe=Get from CANoe
      settings: AttributesFormatString=%<nsName>::%<sysVarName>  SourceProductName=Vector CANoe
  Val_OverRide_Batt_DischargePowerLim_5s : canoelib/CANoe I//O/System Variable Input  nsName=HIL_Interface  sysVarName=CAN_OverRide::BMS::x109_BMS_HV_10::Batt_DischargePowerLim_5s::Val_OverRide_Batt_DischargePowerLim_5s  arrayIndex=-1  editSampleTime=0.001  rawValue=Default  dataType=Default  dataTypeDB=unknown  hasEncoding=off  dataTypeCANoe=Get from CANoe
      settings: AttributesFormatString=%<nsName>::%<sysVarName>  SourceProductName=Vector CANoe
  Val_OverRide_Batt_EnergyAvailable : canoelib/CANoe I//O/System Variable Input  nsName=HIL_Interface  sysVarName=CAN_OverRide::BMS::xCE_BMS_HV_06::Batt_EnergyAvailable::Val_OverRide_Batt_EnergyAvailable  arrayIndex=-1  editSampleTime=0.001  rawValue=Default  dataType=Default  dataTypeDB=unknown  hasEncoding=off  dataTypeCANoe=Get from CANoe
      settings: AttributesFormatString=%<nsName>::%<sysVarName>  SourceProductName=Vector CANoe
  Val_OverRide_Batt_Equity_SoC_Displayed : canoelib/CANoe I//O/System Variable Input  nsName=HIL_Interface  sysVarName=CAN_OverRide::BMS::xC9_BMS_HV_01_Status::Batt_Equity_SoC_Displayed::Val_OverRide_Batt_Equity_SoC_Displayed  arrayIndex=-1  editSampleTime=0.001  rawValue=Default  dataType=Default  dataTypeDB=unknown  hasEncoding=off  dataTypeCANoe=Get from CANoe
      settings: AttributesFormatString=%<nsName>::%<sysVarName>  SourceProductName=Vector CANoe
  Val_OverRide_Batt_FaultActive_FR4 : canoelib/CANoe I//O/System Variable Input  nsName=HIL_Interface  sysVarName=CAN_OverRide::BMS::x110_BMS_HV_09::Batt_FaultActive_FR4::Val_OverRide_Batt_FaultActive_FR4  arrayIndex=-1  editSampleTime=0.001  rawValue=Default  dataType=Default  dataTypeDB=unknown  hasEncoding=off  dataTypeCANoe=Get from CANoe
      settings: AttributesFormatString=%<nsName>::%<sysVarName>  SourceProductName=Vector CANoe
  Val_OverRide_Batt_Fault_FR0 : canoelib/CANoe I//O/System Variable Input  nsName=HIL_Interface  sysVarName=CAN_OverRide::BMS::xC9_BMS_HV_01_Status::Batt_Fault_FR0::Val_OverRide_Batt_Fault_FR0  arrayIndex=-1  editSampleTime=0.001  rawValue=Default  dataType=Default  dataTypeDB=unknown  hasEncoding=off  dataTypeCANoe=Get from CANoe
      settings: AttributesFormatString=%<nsName>::%<sysVarName>  SourceProductName=Vector CANoe
  Val_OverRide_Batt_Fault_FR1 : canoelib/CANoe I//O/System Variable Input  nsName=HIL_Interface  sysVarName=CAN_OverRide::BMS::xC9_BMS_HV_01_Status::Batt_Fault_FR1::Val_OverRide_Batt_Fault_FR1  arrayIndex=-1  editSampleTime=0.001  rawValue=Default  dataType=Default  dataTypeDB=unknown  hasEncoding=off  dataTypeCANoe=Get from CANoe
      settings: AttributesFormatString=%<nsName>::%<sysVarName>  SourceProductName=Vector CANoe
  Val_OverRide_Batt_Fault_FR2 : canoelib/CANoe I//O/System Variable Input  nsName=HIL_Interface  sysVarName=CAN_OverRide::BMS::xC9_BMS_HV_01_Status::Batt_Fault_FR2::Val_OverRide_Batt_Fault_FR2  arrayIndex=-1  editSampleTime=0.001  rawValue=Default  dataType=Default  dataTypeDB=unknown  hasEncoding=off  dataTypeCANoe=Get from CANoe
      settings: AttributesFormatString=%<nsName>::%<sysVarName>  SourceProductName=Vector CANoe
  Val_OverRide_Batt_Fault_FR3 : canoelib/CANoe I//O/System Variable Input  nsName=HIL_Interface  sysVarName=CAN_OverRide::BMS::xC9_BMS_HV_01_Status::Batt_Fault_FR3::Val_OverRide_Batt_Fault_FR3  arrayIndex=-1  editSampleTime=0.001  rawValue=Default  dataType=Default  dataTypeDB=unknown  hasEncoding=off  dataTypeCANoe=Get from CANoe
      settings: AttributesFormatString=%<nsName>::%<sysVarName>  SourceProductName=Vector CANoe
  Val_OverRide_Batt_Fault_FR4 : canoelib/CANoe I//O/System Variable Input  nsName=HIL_Interface  sysVarName=CAN_OverRide::BMS::xC9_BMS_HV_01_Status::Batt_Fault_FR4::Val_OverRide_Batt_Fault_FR4  arrayIndex=-1  editSampleTime=0.001  rawValue=Default  dataType=Default  dataTypeDB=unknown  hasEncoding=off  dataTypeCANoe=Get from CANoe
      settings: AttributesFormatString=%<nsName>::%<sysVarName>  SourceProductName=Vector CANoe
  Val_OverRide_Batt_Fault_FR5 : canoelib/CANoe I//O/System Variable Input  nsName=HIL_Interface  sysVarName=CAN_OverRide::BMS::xC9_BMS_HV_01_Status::Batt_Fault_FR5::Val_OverRide_Batt_Fault_FR5  arrayIndex=-1  editSampleTime=0.001  rawValue=Default  dataType=Default  dataTypeDB=unknown  hasEncoding=off  dataTypeCANoe=Get from CANoe
      settings: AttributesFormatString=%<nsName>::%<sysVarName>  SourceProductName=Vector CANoe
  Val_OverRide_Batt_Fault_FR6 : canoelib/CANoe I//O/System Variable Input  nsName=HIL_Interface  sysVarName=CAN_OverRide::BMS::xC9_BMS_HV_01_Status::Batt_Fault_FR6::Val_OverRide_Batt_Fault_FR6  arrayIndex=-1  editSampleTime=0.001  rawValue=Default  dataType=Default  dataTypeDB=unknown  hasEncoding=off  dataTypeCANoe=Get from CANoe
      settings: AttributesFormatString=%<nsName>::%<sysVarName>  SourceProductName=Vector CANoe
  Val_OverRide_Batt_Fault_FR7 : canoelib/CANoe I//O/System Variable Input  nsName=HIL_Interface  sysVarName=CAN_OverRide::BMS::xC9_BMS_HV_01_Status::Batt_Fault_FR7::Val_OverRide_Batt_Fault_FR7  arrayIndex=-1  editSampleTime=0.001  rawValue=Default  dataType=Default  dataTypeDB=unknown  hasEncoding=off  dataTypeCANoe=Get from CANoe
      settings: AttributesFormatString=%<nsName>::%<sysVarName>  SourceProductName=Vector CANoe
  Val_OverRide_Batt_HVILFault : canoelib/CANoe I//O/System Variable Input  nsName=HIL_Interface  sysVarName=CAN_OverRide::BMS::xC9_BMS_HV_01_Status::Batt_HVILFault::Val_OverRide_Batt_HVILFault  arrayIndex=-1  editSampleTime=0.001  rawValue=Default  dataType=Default  dataTypeDB=unknown  hasEncoding=off  dataTypeCANoe=Get from CANoe
      settings: AttributesFormatString=%<nsName>::%<sysVarName>  SourceProductName=Vector CANoe
  Val_OverRide_Batt_InvOutVoltage : canoelib/CANoe I//O/System Variable Input  nsName=HIL_Interface  sysVarName=CAN_OverRide::BMS::xCC_BMS_HV_04_ContactorStatus::Batt_InvOutVoltage::Val_OverRide_Batt_InvOutVoltage  arrayIndex=-1  editSampleTime=0.001  rawValue=Default  dataType=Default  dataTypeDB=unknown  hasEncoding=off  dataTypeCANoe=Get from CANoe
      settings: AttributesFormatString=%<nsName>::%<sysVarName>  SourceProductName=Vector CANoe
  Val_OverRide_Batt_Isolation1OnOffStatus : canoelib/CANoe I//O/System Variable Input  nsName=HIL_Interface  sysVarName=CAN_OverRide::BMS::xC9_BMS_HV_01_Status::Batt_Isolation1OnOffStatus::Val_OverRide_Batt_Isolation1OnOffStatus  arrayIndex=-1  editSampleTime=0.001  rawValue=Default  dataType=Default  dataTypeDB=unknown  hasEncoding=off  dataTypeCANoe=Get from CANoe
      settings: AttributesFormatString=%<nsName>::%<sysVarName>  SourceProductName=Vector CANoe
  Val_OverRide_Batt_Isolation1Res_HighRange : canoelib/CANoe I//O/System Variable Input  nsName=HIL_Interface  sysVarName=CAN_OverRide::BMS::xCE_BMS_HV_06::Batt_Isolation1Res_HighRange::Val_OverRide_Batt_Isolation1Res_HighRange  arrayIndex=-1  editSampleTime=0.001  rawValue=Default  dataType=Default  dataTypeDB=unknown  hasEncoding=off  dataTypeCANoe=Get from CANoe
      settings: AttributesFormatString=%<nsName>::%<sysVarName>  SourceProductName=Vector CANoe
  Val_OverRide_Batt_Isolation1Resistance : canoelib/CANoe I//O/System Variable Input  nsName=HIL_Interface  sysVarName=CAN_OverRide::BMS::xCE_BMS_HV_06::Batt_Isolation1Resistance::Val_OverRide_Batt_Isolation1Resistance  arrayIndex=-1  editSampleTime=0.001  rawValue=Default  dataType=Default  dataTypeDB=unknown  hasEncoding=off  dataTypeCANoe=Get from CANoe
      settings: AttributesFormatString=%<nsName>::%<sysVarName>  SourceProductName=Vector CANoe
  Val_OverRide_Batt_Isolation1Status : canoelib/CANoe I//O/System Variable Input  nsName=HIL_Interface  sysVarName=CAN_OverRide::BMS::xC9_BMS_HV_01_Status::Batt_Isolation1Status::Val_OverRide_Batt_Isolation1Status  arrayIndex=-1  editSampleTime=0.001  rawValue=Default  dataType=Default  dataTypeDB=unknown  hasEncoding=off  dataTypeCANoe=Get from CANoe
      settings: AttributesFormatString=%<nsName>::%<sysVarName>  SourceProductName=Vector CANoe
  Val_OverRide_Batt_Isolation2OnOffStatus : canoelib/CANoe I//O/System Variable Input  nsName=HIL_Interface  sysVarName=CAN_OverRide::BMS::xC9_BMS_HV_01_Status::Batt_Isolation2OnOffStatus::Val_OverRide_Batt_Isolation2OnOffStatus  arrayIndex=-1  editSampleTime=0.001  rawValue=Default  dataType=Default  dataTypeDB=unknown  hasEncoding=off  dataTypeCANoe=Get from CANoe
      settings: AttributesFormatString=%<nsName>::%<sysVarName>  SourceProductName=Vector CANoe
  Val_OverRide_Batt_Isolation2Status : canoelib/CANoe I//O/System Variable Input  nsName=HIL_Interface  sysVarName=CAN_OverRide::BMS::xC9_BMS_HV_01_Status::Batt_Isolation2Status::Val_OverRide_Batt_Isolation2Status  arrayIndex=-1  editSampleTime=0.001  rawValue=Default  dataType=Default  dataTypeDB=unknown  hasEncoding=off  dataTypeCANoe=Get from CANoe
      settings: AttributesFormatString=%<nsName>::%<sysVarName>  SourceProductName=Vector CANoe
  Val_OverRide_Batt_LVBackupBattVoltage : canoelib/CANoe I//O/System Variable Input  nsName=HIL_Interface  sysVarName=CAN_OverRide::BMS::xCF_BMS_HV_07_Thermal::Batt_LVBackupBattVoltage::Val_OverRide_Batt_LVBackupBattVoltage  arrayIndex=-1  editSampleTime=0.001  rawValue=Default  dataType=Default  dataTypeDB=unknown  hasEncoding=off  dataTypeCANoe=Get from CANoe
      settings: AttributesFormatString=%<nsName>::%<sysVarName>  SourceProductName=Vector CANoe
  Val_OverRide_Batt_LVVoltage : canoelib/CANoe I//O/System Variable Input  nsName=HIL_Interface  sysVarName=CAN_OverRide::BMS::xCE_BMS_HV_06::Batt_LVVoltage::Val_OverRide_Batt_LVVoltage  arrayIndex=-1  editSampleTime=0.001  rawValue=Default  dataType=Default  dataTypeDB=unknown  hasEncoding=off  dataTypeCANoe=Get from CANoe
      settings: AttributesFormatString=%<nsName>::%<sysVarName>  SourceProductName=Vector CANoe
  Val_OverRide_Batt_LoggerPercent : canoelib/CANoe I//O/System Variable Input  nsName=HIL_Interface  sysVarName=CAN_OverRide::BMS::x110_BMS_HV_09::Batt_LoggerPercent::Val_OverRide_Batt_LoggerPercent  arrayIndex=-1  editSampleTime=0.001  rawValue=Default  dataType=Default  dataTypeDB=unknown  hasEncoding=off  dataTypeCANoe=Get from CANoe
      settings: AttributesFormatString=%<nsName>::%<sysVarName>  SourceProductName=Vector CANoe
  Val_OverRide_Batt_MainContactorStatus : canoelib/CANoe I//O/System Variable Input  nsName=HIL_Interface  sysVarName=CAN_OverRide::BMS::xCC_BMS_HV_04_ContactorStatus::Batt_MainContactorStatus::Val_OverRide_Batt_MainContactorStatus  arrayIndex=-1  editSampleTime=0.001  rawValue=Default  dataType=Default  dataTypeDB=unknown  hasEncoding=off  dataTypeCANoe=Get from CANoe
      settings: AttributesFormatString=%<nsName>::%<sysVarName>  SourceProductName=Vector CANoe
  Val_OverRide_Batt_MaxCellTemperature : canoelib/CANoe I//O/System Variable Input  nsName=HIL_Interface  sysVarName=CAN_OverRide::BMS::xCD_BMS_HV_05_CellParam::Batt_MaxCellTemperature::Val_OverRide_Batt_MaxCellTemperature  arrayIndex=-1  editSampleTime=0.001  rawValue=Default  dataType=Default  dataTypeDB=unknown  hasEncoding=off  dataTypeCANoe=Get from CANoe
      settings: AttributesFormatString=%<nsName>::%<sysVarName>  SourceProductName=Vector CANoe
  Val_OverRide_Batt_MaxCellVoltage : canoelib/CANoe I//O/System Variable Input  nsName=HIL_Interface  sysVarName=CAN_OverRide::BMS::xCD_BMS_HV_05_CellParam::Batt_MaxCellVoltage::Val_OverRide_Batt_MaxCellVoltage  arrayIndex=-1  editSampleTime=0.001  rawValue=Default  dataType=Default  dataTypeDB=unknown  hasEncoding=off  dataTypeCANoe=Get from CANoe
      settings: AttributesFormatString=%<nsName>::%<sysVarName>  SourceProductName=Vector CANoe
  Val_OverRide_Batt_MaxSOC : canoelib/CANoe I//O/System Variable Input  nsName=HIL_Interface  sysVarName=CAN_OverRide::BMS::x110_BMS_HV_09::Batt_MaxSOC::Val_OverRide_Batt_MaxSOC  arrayIndex=-1  editSampleTime=0.001  rawValue=Default  dataType=Default  dataTypeDB=unknown  hasEncoding=off  dataTypeCANoe=Get from CANoe
      settings: AttributesFormatString=%<nsName>::%<sysVarName>  SourceProductName=Vector CANoe
  Val_OverRide_Batt_MinCellTemperature : canoelib/CANoe I//O/System Variable Input  nsName=HIL_Interface  sysVarName=CAN_OverRide::BMS::xCD_BMS_HV_05_CellParam::Batt_MinCellTemperature::Val_OverRide_Batt_MinCellTemperature  arrayIndex=-1  editSampleTime=0.001  rawValue=Default  dataType=Default  dataTypeDB=unknown  hasEncoding=off  dataTypeCANoe=Get from CANoe
      settings: AttributesFormatString=%<nsName>::%<sysVarName>  SourceProductName=Vector CANoe
  Val_OverRide_Batt_MinCellVoltage : canoelib/CANoe I//O/System Variable Input  nsName=HIL_Interface  sysVarName=CAN_OverRide::BMS::xCD_BMS_HV_05_CellParam::Batt_MinCellVoltage::Val_OverRide_Batt_MinCellVoltage  arrayIndex=-1  editSampleTime=0.001  rawValue=Default  dataType=Default  dataTypeDB=unknown  hasEncoding=off  dataTypeCANoe=Get from CANoe
      settings: AttributesFormatString=%<nsName>::%<sysVarName>  SourceProductName=Vector CANoe
  Val_OverRide_Batt_MinSOC : canoelib/CANoe I//O/System Variable Input  nsName=HIL_Interface  sysVarName=CAN_OverRide::BMS::xC9_BMS_HV_01_Status::Batt_MinSOC::Val_OverRide_Batt_MinSOC  arrayIndex=-1  editSampleTime=0.001  rawValue=Default  dataType=Default  dataTypeDB=unknown  hasEncoding=off  dataTypeCANoe=Get from CANoe
      settings: AttributesFormatString=%<nsName>::%<sysVarName>  SourceProductName=Vector CANoe
  Val_OverRide_Batt_ReadyforBoostCharge : canoelib/CANoe I//O/System Variable Input  nsName=HIL_Interface  sysVarName=CAN_OverRide::BMS::xD2_BMS_HV_08::Batt_ReadyforBoostCharge::Val_OverRide_Batt_ReadyforBoostCharge  arrayIndex=-1  editSampleTime=0.001  rawValue=Default  dataType=Default  dataTypeDB=unknown  hasEncoding=off  dataTypeCANoe=Get from CANoe
      settings: AttributesFormatString=%<nsName>::%<sysVarName>  SourceProductName=Vector CANoe
  Val_OverRide_Batt_ReadytoTurnOnHV : canoelib/CANoe I//O/System Variable Input  nsName=HIL_Interface  sysVarName=CAN_OverRide::BMS::xC9_BMS_HV_01_Status::Batt_ReadytoTurnOnHV::Val_OverRide_Batt_ReadytoTurnOnHV  arrayIndex=-1  editSampleTime=0.001  rawValue=Default  dataType=Default  dataTypeDB=unknown  hasEncoding=off  dataTypeCANoe=Get from CANoe
      settings: AttributesFormatString=%<nsName>::%<sysVarName>  SourceProductName=Vector CANoe
  Val_OverRide_Batt_RegenPowerLim : canoelib/CANoe I//O/System Variable Input  nsName=HIL_Interface  sysVarName=CAN_OverRide::BMS::xCB_BMS_HV_03_BatteryLimits::Batt_RegenPowerLim::Val_OverRide_Batt_RegenPowerLim  arrayIndex=-1  editSampleTime=0.001  rawValue=Default  dataType=Default  dataTypeDB=unknown  hasEncoding=off  dataTypeCANoe=Get from CANoe
      settings: AttributesFormatString=%<nsName>::%<sysVarName>  SourceProductName=Vector CANoe
  Val_OverRide_Batt_RegenPowerLim_2s : canoelib/CANoe I//O/System Variable Input  nsName=HIL_Interface  sysVarName=CAN_OverRide::BMS::x109_BMS_HV_10::Batt_RegenPowerLim_2s::Val_OverRide_Batt_RegenPowerLim_2s  arrayIndex=-1  editSampleTime=0.001  rawValue=Default  dataType=Default  dataTypeDB=unknown  hasEncoding=off  dataTypeCANoe=Get from CANoe
      settings: AttributesFormatString=%<nsName>::%<sysVarName>  SourceProductName=Vector CANoe
  Val_OverRide_Batt_RegenPowerLim_5s : canoelib/CANoe I//O/System Variable Input  nsName=HIL_Interface  sysVarName=CAN_OverRide::BMS::x109_BMS_HV_10::Batt_RegenPowerLim_5s::Val_OverRide_Batt_RegenPowerLim_5s  arrayIndex=-1  editSampleTime=0.001  rawValue=Default  dataType=Default  dataTypeDB=unknown  hasEncoding=off  dataTypeCANoe=Get from CANoe
      settings: AttributesFormatString=%<nsName>::%<sysVarName>  SourceProductName=Vector CANoe
  Val_OverRide_Batt_SafetyLightStatGreenHV : canoelib/CANoe I//O/System Variable Input  nsName=HIL_Interface  sysVarName=CAN_OverRide::BMS::xD2_BMS_HV_08::Batt_SafetyLightStatGreenHV::Val_OverRide_Batt_SafetyLightStatGreenHV  arrayIndex=-1  editSampleTime=0.001  rawValue=Default  dataType=Default  dataTypeDB=unknown  hasEncoding=off  dataTypeCANoe=Get from CANoe
      settings: AttributesFormatString=%<nsName>::%<sysVarName>  SourceProductName=Vector CANoe
  Val_OverRide_Batt_SafetyLightStatRedHV : canoelib/CANoe I//O/System Variable Input  nsName=HIL_Interface  sysVarName=CAN_OverRide::BMS::xD2_BMS_HV_08::Batt_SafetyLightStatRedHV::Val_OverRide_Batt_SafetyLightStatRedHV  arrayIndex=-1  editSampleTime=0.001  rawValue=Default  dataType=Default  dataTypeDB=unknown  hasEncoding=off  dataTypeCANoe=Get from CANoe
      settings: AttributesFormatString=%<nsName>::%<sysVarName>  SourceProductName=Vector CANoe
  Val_OverRide_Batt_SerialNumber : canoelib/CANoe I//O/System Variable Input  nsName=HIL_Interface  sysVarName=CAN_OverRide::BMS::x112_BMS_HV_12::Batt_SerialNumber::Val_OverRide_Batt_SerialNumber  arrayIndex=-1  editSampleTime=0.001  rawValue=Default  dataType=Default  dataTypeDB=unknown  hasEncoding=off  dataTypeCANoe=Get from CANoe
      settings: AttributesFormatString=%<nsName>::%<sysVarName>  SourceProductName=Vector CANoe
  Val_OverRide_Batt_ThermalRequest : canoelib/CANoe I//O/System Variable Input  nsName=HIL_Interface  sysVarName=CAN_OverRide::BMS::xCF_BMS_HV_07_Thermal::Batt_ThermalRequest::Val_OverRide_Batt_ThermalRequest  arrayIndex=-1  editSampleTime=0.001  rawValue=Default  dataType=Default  dataTypeDB=unknown  hasEncoding=off  dataTypeCANoe=Get from CANoe
      settings: AttributesFormatString=%<nsName>::%<sysVarName>  SourceProductName=Vector CANoe
  Val_OverRide_Batt_UserSOC : canoelib/CANoe I//O/System Variable Input  nsName=HIL_Interface  sysVarName=CAN_OverRide::BMS::xC9_BMS_HV_01_Status::Batt_UserSOC::Val_OverRide_Batt_UserSOC  arrayIndex=-1  editSampleTime=0.001  rawValue=Default  dataType=Default  dataTypeDB=unknown  hasEncoding=off  dataTypeCANoe=Get from CANoe
      settings: AttributesFormatString=%<nsName>::%<sysVarName>  SourceProductName=Vector CANoe
  Val_OverRide_Batt_Voltage : canoelib/CANoe I//O/System Variable Input  nsName=HIL_Interface  sysVarName=CAN_OverRide::BMS::xCA_BMS_HV_02_HVParameter::Batt_Voltage::Val_OverRide_Batt_Voltage  arrayIndex=-1  editSampleTime=0.001  rawValue=Default  dataType=Default  dataTypeDB=unknown  hasEncoding=off  dataTypeCANoe=Get from CANoe
      settings: AttributesFormatString=%<nsName>::%<sysVarName>  SourceProductName=Vector CANoe
  Val_OverRide_CIM_ChargePlugLockStatusHV : canoelib/CANoe I//O/System Variable Input  nsName=HIL_Interface  sysVarName=CAN_OverRide::BMS::x12D_CIM_HV_01::CIM_ChargePlugLockStatusHV::Val_OverRide_CIM_ChargePlugLockStatusHV  arrayIndex=-1  editSampleTime=0.001  rawValue=Default  dataType=Default  dataTypeDB=unknown  hasEncoding=off  dataTypeCANoe=Get from CANoe
      settings: AttributesFormatString=%<nsName>::%<sysVarName>  SourceProductName=Vector CANoe
  Val_OverRide_CIM_ChargeStatusHV : canoelib/CANoe I//O/System Variable Input  nsName=HIL_Interface  sysVarName=CAN_OverRide::BMS::x12D_CIM_HV_01::CIM_ChargeStatusHV::Val_OverRide_CIM_ChargeStatusHV  arrayIndex=-1  editSampleTime=0.001  rawValue=Default  dataType=Default  dataTypeDB=unknown  hasEncoding=off  dataTypeCANoe=Get from CANoe
      settings: AttributesFormatString=%<nsName>::%<sysVarName>  SourceProductName=Vector CANoe
  Val_OverRide_CIM_ChargingPlugTypeHV : canoelib/CANoe I//O/System Variable Input  nsName=HIL_Interface  sysVarName=CAN_OverRide::BMS::x12D_CIM_HV_01::CIM_ChargingPlugTypeHV::Val_OverRide_CIM_ChargingPlugTypeHV  arrayIndex=-1  editSampleTime=0.001  rawValue=Default  dataType=Default  dataTypeDB=unknown  hasEncoding=off  dataTypeCANoe=Get from CANoe
      settings: AttributesFormatString=%<nsName>::%<sysVarName>  SourceProductName=Vector CANoe
  Val_OverRide_CIM_PlugPresentHV : canoelib/CANoe I//O/System Variable Input  nsName=HIL_Interface  sysVarName=CAN_OverRide::BMS::x12D_CIM_HV_01::CIM_PlugPresentHV::Val_OverRide_CIM_PlugPresentHV  arrayIndex=-1  editSampleTime=0.001  rawValue=Default  dataType=Default  dataTypeDB=unknown  hasEncoding=off  dataTypeCANoe=Get from CANoe
      settings: AttributesFormatString=%<nsName>::%<sysVarName>  SourceProductName=Vector CANoe
  En_OverRide_Batt_AncOutVoltage_port : Outport
  Val_OverRide_Batt_AncOutVoltage_port : Outport  Port=2
  En_OverRide_Batt_ChargeContactorStatus_port : Outport  Port=3
  Val_OverRide_Batt_ChargeContactorStatus_port : Outport  Port=4
  En_OverRide_Batt_InvOutVoltage_port : Outport  Port=5
  Val_OverRide_Batt_InvOutVoltage_port : Outport  Port=6
  En_OverRide_Batt_MainContactorStatus_port : Outport  Port=7
  Val_OverRide_Batt_MainContactorStatus_port : Outport  Port=8
  En_OverRide_Batt_BalancingRequired_port : Outport  Port=9
  Val_OverRide_Batt_BalancingRequired_port : Outport  Port=10
  En_OverRide_Batt_BMSStatus_port : Outport  Port=11
  Val_OverRide_Batt_BMSStatus_port : Outport  Port=12
  En_OverRide_Batt_Equity_SoC_Displayed_port : Outport  Port=13
  Val_OverRide_Batt_Equity_SoC_Displayed_port : Outport  Port=14
  En_OverRide_Batt_Fault_FR0_port : Outport  Port=15
  Val_OverRide_Batt_Fault_FR0_port : Outport  Port=16
  En_OverRide_Batt_Fault_FR1_port : Outport  Port=17
  Val_OverRide_Batt_Fault_FR1_port : Outport  Port=18
  En_OverRide_Batt_Fault_FR2_port : Outport  Port=19
  Val_OverRide_Batt_Fault_FR2_port : Outport  Port=20
  En_OverRide_Batt_Fault_FR3_port : Outport  Port=21
  Val_OverRide_Batt_Fault_FR3_port : Outport  Port=22
  En_OverRide_Batt_Fault_FR4_port : Outport  Port=23
  Val_OverRide_Batt_Fault_FR4_port : Outport  Port=24
  En_OverRide_Batt_Fault_FR5_port : Outport  Port=25
  Val_OverRide_Batt_Fault_FR5_port : Outport  Port=26
  En_OverRide_Batt_Fault_FR6_port : Outport  Port=27
  Val_OverRide_Batt_Fault_FR6_port : Outport  Port=28
  En_OverRide_Batt_Fault_FR7_port : Outport  Port=29
  Val_OverRide_Batt_Fault_FR7_port : Outport  Port=30
  En_OverRide_Batt_HVILFault_port : Outport  Port=31
  Val_OverRide_Batt_HVILFault_port : Outport  Port=32
  En_OverRide_Batt_Isolation1OnOffStatus_port : Outport  Port=33
  Val_OverRide_Batt_Isolation1OnOffStatus_port : Outport  Port=34
  En_OverRide_Batt_Isolation1Status_port : Outport  Port=35
  Val_OverRide_Batt_Isolation1Status_port : Outport  Port=36
  En_OverRide_Batt_Isolation2OnOffStatus_port : Outport  Port=37
  Val_OverRide_Batt_Isolation2OnOffStatus_port : Outport  Port=38
  En_OverRide_Batt_Isolation2Status_port : Outport  Port=39
  Val_OverRide_Batt_Isolation2Status_port : Outport  Port=40
  En_OverRide_Batt_MinSOC_port : Outport  Port=41
  Val_OverRide_Batt_MinSOC_port : Outport  Port=42
  En_OverRide_Batt_ReadytoTurnOnHV_port : Outport  Port=43
  Val_OverRide_Batt_ReadytoTurnOnHV_port : Outport  Port=44
  En_OverRide_Batt_UserSOC_port : Outport  Port=45
  Val_OverRide_Batt_UserSOC_port : Outport  Port=46
  En_OverRide_BMS_AliveCounter1_port : Outport  Port=47
  Val_OverRide_BMS_AliveCounter1_port : Outport  Port=48
  En_OverRide_Batt_BoostChargeActive_port : Outport  Port=49
  Val_OverRide_Batt_BoostChargeActive_port : Outport  Port=50
  En_OverRide_Batt_DischEnergyThroughput_port : Outport  Port=51
  Val_OverRide_Batt_DischEnergyThroughput_port : Outport  Port=52
  En_OverRide_Batt_ReadyforBoostCharge_port : Outport  Port=53
  Val_OverRide_Batt_ReadyforBoostCharge_port : Outport  Port=54
  En_OverRide_Batt_SafetyLightStatGreenHV_port : Outport  Port=55
  Val_OverRide_Batt_SafetyLightStatGreenHV_port : Outport  Port=56
  En_OverRide_Batt_SafetyLightStatRedHV_port : Outport  Port=57
  Val_OverRide_Batt_SafetyLightStatRedHV_port : Outport  Port=58
  En_OverRide_Batt_ClearFault_Code_port : Outport  Port=59
  Val_OverRide_Batt_ClearFault_Code_port : Outport  Port=60
  En_OverRide_Batt_ClearFault_KeyMatched_port : Outport  Port=61
  Val_OverRide_Batt_ClearFault_KeyMatched_port : Outport  Port=62
  En_OverRide_Batt_FaultActive_FR4_port : Outport  Port=63
  Val_OverRide_Batt_FaultActive_FR4_port : Outport  Port=64
  En_OverRide_Batt_LoggerPercent_port : Outport  Port=65
  Val_OverRide_Batt_LoggerPercent_port : Outport  Port=66
  En_OverRide_Batt_MaxSOC_port : Outport  Port=67
  Val_OverRide_Batt_MaxSOC_port : Outport  Port=68
  En_OverRide_BMS_LoggingFull_port : Outport  Port=69
  Val_OverRide_BMS_LoggingFull_port : Outport  Port=70
  En_OverRide_Batt_Coolant_IN_Pressure_port : Outport  Port=71
  Val_OverRide_Batt_Coolant_IN_Pressure_port : Outport  Port=72
  En_OverRide_Batt_Coolant_IN_Temp_port : Outport  Port=73
  Val_OverRide_Batt_Coolant_IN_Temp_port : Outport  Port=74
  En_OverRide_Batt_Coolant_OUT_Pressure_port : Outport  Port=75
  Val_OverRide_Batt_Coolant_OUT_Pressure_port : Outport  Port=76
  En_OverRide_Batt_Coolant_OUT_Temp_port : Outport  Port=77
  Val_OverRide_Batt_Coolant_OUT_Temp_port : Outport  Port=78
  En_OverRide_Batt_LVBackupBattVoltage_port : Outport  Port=79
  Val_OverRide_Batt_LVBackupBattVoltage_port : Outport  Port=80
  En_OverRide_Batt_ThermalRequest_port : Outport  Port=81
  Val_OverRide_Batt_ThermalRequest_port : Outport  Port=82
  En_OverRide_Batt_Current_port : Outport  Port=83
  Val_OverRide_Batt_Current_port : Outport  Port=84
  En_OverRide_Batt_Voltage_port : Outport  Port=85
  Val_OverRide_Batt_Voltage_port : Outport  Port=86
  En_OverRide_BMS_AliveCounter2_port : Outport  Port=87
  Val_OverRide_BMS_AliveCounter2_port : Outport  Port=88
  En_OverRide_Batt_DischargePowerLim_port : Outport  Port=89
  Val_OverRide_Batt_DischargePowerLim_port : Outport  Port=90
  En_OverRide_Batt_RegenPowerLim_port : Outport  Port=91
  Val_OverRide_Batt_RegenPowerLim_port : Outport  Port=92
  En_OverRide_BMS_AliveCounter3_port : Outport  Port=93
  Val_OverRide_BMS_AliveCounter3_port : Outport  Port=94
  En_OverRide_Batt_DischargePowerLim_2s_port : Outport  Port=95
  Val_OverRide_Batt_DischargePowerLim_2s_port : Outport  Port=96
  En_OverRide_Batt_DischargePowerLim_5s_port : Outport  Port=97
  Val_OverRide_Batt_DischargePowerLim_5s_port : Outport  Port=98
  En_OverRide_Batt_RegenPowerLim_2s_port : Outport  Port=99
  Val_OverRide_Batt_RegenPowerLim_2s_port : Outport  Port=100
  En_OverRide_Batt_RegenPowerLim_5s_port : Outport  Port=101
  Val_OverRide_Batt_RegenPowerLim_5s_port : Outport  Port=102
  En_OverRide_Batt_EnergyAvailable_port : Outport  Port=103
  Val_OverRide_Batt_EnergyAvailable_port : Outport  Port=104
  En_OverRide_Batt_Isolation1Res_HighRange_port : Outport  Port=105
  Val_OverRide_Batt_Isolation1Res_HighRange_port : Outport  Port=106
  En_OverRide_Batt_Isolation1Resistance_port : Outport  Port=107
  Val_OverRide_Batt_Isolation1Resistance_port : Outport  Port=108
  En_OverRide_Batt_LVVoltage_port : Outport  Port=109
  Val_OverRide_Batt_LVVoltage_port : Outport  Port=110
  En_OverRide_Batt_MaxCellTemperature_port : Outport  Port=111
  Val_OverRide_Batt_MaxCellTemperature_port : Outport  Port=112
  En_OverRide_Batt_MaxCellVoltage_port : Outport  Port=113
  Val_OverRide_Batt_MaxCellVoltage_port : Outport  Port=114
  En_OverRide_Batt_MinCellTemperature_port : Outport  Port=115
  Val_OverRide_Batt_MinCellTemperature_port : Outport  Port=116
  En_OverRide_Batt_MinCellVoltage_port : Outport  Port=117
  Val_OverRide_Batt_MinCellVoltage_port : Outport  Port=118
  En_OverRide_Batt_SerialNumber_port : Outport  Port=119
  Val_OverRide_Batt_SerialNumber_port : Outport  Port=120
  En_OverRide_BMS_Calibration_info_port : Outport  Port=121
  Val_OverRide_BMS_Calibration_info_port : Outport  Port=122
  En_OverRide_BMS_Software_info_port : Outport  Port=123
  Val_OverRide_BMS_Software_info_port : Outport  Port=124
  En_OverRide_CIM_ChargePlugLockStatusHV_port : Outport  Port=125
  Val_OverRide_CIM_ChargePlugLockStatusHV_port : Outport  Port=126
  En_OverRide_CIM_ChargeStatusHV_port : Outport  Port=127
  Val_OverRide_CIM_ChargeStatusHV_port : Outport  Port=128
  En_OverRide_CIM_ChargingPlugTypeHV_port : Outport  Port=129
  Val_OverRide_CIM_ChargingPlugTypeHV_port : Outport  Port=130
  En_OverRide_CIM_PlugPresentHV_port : Outport  Port=131
  Val_OverRide_CIM_PlugPresentHV_port : Outport  Port=132
  wires:
  ? -> ?
  En_OverRide_Batt_AncOutVoltage/1 -> En_OverRide_Batt_AncOutVoltage_port/1
  Val_OverRide_Batt_AncOutVoltage/1 -> Val_OverRide_Batt_AncOutVoltage_port/1
  En_OverRide_Batt_ChargeContactorStatus/1 -> En_OverRide_Batt_ChargeContactorStatus_port/1
  Val_OverRide_Batt_ChargeContactorStatus/1 -> Val_OverRide_Batt_ChargeContactorStatus_port/1
  En_OverRide_Batt_InvOutVoltage/1 -> En_OverRide_Batt_InvOutVoltage_port/1
  Val_OverRide_Batt_InvOutVoltage/1 -> Val_OverRide_Batt_InvOutVoltage_port/1
  En_OverRide_Batt_MainContactorStatus/1 -> En_OverRide_Batt_MainContactorStatus_port/1
  Val_OverRide_Batt_MainContactorStatus/1 -> Val_OverRide_Batt_MainContactorStatus_port/1
  En_OverRide_Batt_BalancingRequired/1 -> En_OverRide_Batt_BalancingRequired_port/1
  Val_OverRide_Batt_BalancingRequired/1 -> Val_OverRide_Batt_BalancingRequired_port/1
  En_OverRide_Batt_BMSStatus/1 -> En_OverRide_Batt_BMSStatus_port/1
  Val_OverRide_Batt_BMSStatus/1 -> Val_OverRide_Batt_BMSStatus_port/1
  En_OverRide_Batt_Equity_SoC_Displayed/1 -> En_OverRide_Batt_Equity_SoC_Displayed_port/1
  Val_OverRide_Batt_Equity_SoC_Displayed/1 -> Val_OverRide_Batt_Equity_SoC_Displayed_port/1
  En_OverRide_Batt_Fault_FR0/1 -> En_OverRide_Batt_Fault_FR0_port/1
  Val_OverRide_Batt_Fault_FR0/1 -> Val_OverRide_Batt_Fault_FR0_port/1
  En_OverRide_Batt_Fault_FR1/1 -> En_OverRide_Batt_Fault_FR1_port/1
  Val_OverRide_Batt_Fault_FR1/1 -> Val_OverRide_Batt_Fault_FR1_port/1
  En_OverRide_Batt_Fault_FR2/1 -> En_OverRide_Batt_Fault_FR2_port/1
  Val_OverRide_Batt_Fault_FR2/1 -> Val_OverRide_Batt_Fault_FR2_port/1
  En_OverRide_Batt_Fault_FR3/1 -> En_OverRide_Batt_Fault_FR3_port/1
  Val_OverRide_Batt_Fault_FR3/1 -> Val_OverRide_Batt_Fault_FR3_port/1
  En_OverRide_Batt_Fault_FR4/1 -> En_OverRide_Batt_Fault_FR4_port/1
  Val_OverRide_Batt_Fault_FR4/1 -> Val_OverRide_Batt_Fault_FR4_port/1
  En_OverRide_Batt_Fault_FR5/1 -> En_OverRide_Batt_Fault_FR5_port/1
  Val_OverRide_Batt_Fault_FR5/1 -> Val_OverRide_Batt_Fault_FR5_port/1
  En_OverRide_Batt_Fault_FR6/1 -> En_OverRide_Batt_Fault_FR6_port/1
  Val_OverRide_Batt_Fault_FR6/1 -> Val_OverRide_Batt_Fault_FR6_port/1
  En_OverRide_Batt_Fault_FR7/1 -> En_OverRide_Batt_Fault_FR7_port/1
  Val_OverRide_Batt_Fault_FR7/1 -> Val_OverRide_Batt_Fault_FR7_port/1
  En_OverRide_Batt_HVILFault/1 -> En_OverRide_Batt_HVILFault_port/1
  Val_OverRide_Batt_HVILFault/1 -> Val_OverRide_Batt_HVILFault_port/1
  En_OverRide_Batt_Isolation1OnOffStatus/1 -> En_OverRide_Batt_Isolation1OnOffStatus_port/1
  Val_OverRide_Batt_Isolation1OnOffStatus/1 -> Val_OverRide_Batt_Isolation1OnOffStatus_port/1
  En_OverRide_Batt_Isolation1Status/1 -> En_OverRide_Batt_Isolation1Status_port/1
  Val_OverRide_Batt_Isolation1Status/1 -> Val_OverRide_Batt_Isolation1Status_port/1
  En_OverRide_Batt_Isolation2OnOffStatus/1 -> En_OverRide_Batt_Isolation2OnOffStatus_port/1
  Val_OverRide_Batt_Isolation2OnOffStatus/1 -> Val_OverRide_Batt_Isolation2OnOffStatus_port/1
  En_OverRide_Batt_Isolation2Status/1 -> En_OverRide_Batt_Isolation2Status_port/1
  Val_OverRide_Batt_Isolation2Status/1 -> Val_OverRide_Batt_Isolation2Status_port/1
  En_OverRide_Batt_MinSOC/1 -> En_OverRide_Batt_MinSOC_port/1
  Val_OverRide_Batt_MinSOC/1 -> Val_OverRide_Batt_MinSOC_port/1
  En_OverRide_Batt_ReadytoTurnOnHV/1 -> En_OverRide_Batt_ReadytoTurnOnHV_port/1
  Val_OverRide_Batt_ReadytoTurnOnHV/1 -> Val_OverRide_Batt_ReadytoTurnOnHV_port/1
  En_OverRide_Batt_UserSOC/1 -> En_OverRide_Batt_UserSOC_port/1
  Val_OverRide_Batt_UserSOC/1 -> Val_OverRide_Batt_UserSOC_port/1
  En_OverRide_BMS_AliveCounter1/1 -> En_OverRide_BMS_AliveCounter1_port/1
  Val_OverRide_BMS_AliveCounter1/1 -> Val_OverRide_BMS_AliveCounter1_port/1
  En_OverRide_Batt_BoostChargeActive/1 -> En_OverRide_Batt_BoostChargeActive_port/1
  Val_OverRide_Batt_BoostChargeActive/1 -> Val_OverRide_Batt_BoostChargeActive_port/1
  En_OverRide_Batt_DischEnergyThroughput/1 -> En_OverRide_Batt_DischEnergyThroughput_port/1
  Val_OverRide_Batt_DischEnergyThroughput/1 -> Val_OverRide_Batt_DischEnergyThroughput_port/1
  En_OverRide_Batt_ReadyforBoostCharge/1 -> En_OverRide_Batt_ReadyforBoostCharge_port/1
  Val_OverRide_Batt_ReadyforBoostCharge/1 -> Val_OverRide_Batt_ReadyforBoostCharge_port/1
  En_OverRide_Batt_SafetyLightStatGreenHV/1 -> En_OverRide_Batt_SafetyLightStatGreenHV_port/1
  Val_OverRide_Batt_SafetyLightStatGreenHV/1 -> Val_OverRide_Batt_SafetyLightStatGreenHV_port/1
  En_OverRide_Batt_SafetyLightStatRedHV/1 -> En_OverRide_Batt_SafetyLightStatRedHV_port/1
  Val_OverRide_Batt_SafetyLightStatRedHV/1 -> Val_OverRide_Batt_SafetyLightStatRedHV_port/1
  En_OverRide_Batt_ClearFault_Code/1 -> En_OverRide_Batt_ClearFault_Code_port/1
  Val_OverRide_Batt_ClearFault_Code/1 -> Val_OverRide_Batt_ClearFault_Code_port/1
  En_OverRide_Batt_ClearFault_KeyMatched/1 -> En_OverRide_Batt_ClearFault_KeyMatched_port/1
  Val_OverRide_Batt_ClearFault_KeyMatched/1 -> Val_OverRide_Batt_ClearFault_KeyMatched_port/1
  En_OverRide_Batt_FaultActive_FR4/1 -> En_OverRide_Batt_FaultActive_FR4_port/1
  Val_OverRide_Batt_FaultActive_FR4/1 -> Val_OverRide_Batt_FaultActive_FR4_port/1
  En_OverRide_Batt_LoggerPercent/1 -> En_OverRide_Batt_LoggerPercent_port/1
  Val_OverRide_Batt_LoggerPercent/1 -> Val_OverRide_Batt_LoggerPercent_port/1
  En_OverRide_Batt_MaxSOC/1 -> En_OverRide_Batt_MaxSOC_port/1
  Val_OverRide_Batt_MaxSOC/1 -> Val_OverRide_Batt_MaxSOC_port/1
  En_OverRide_BMS_LoggingFull/1 -> En_OverRide_BMS_LoggingFull_port/1
  Val_OverRide_BMS_LoggingFull/1 -> Val_OverRide_BMS_LoggingFull_port/1
  En_OverRide_Batt_Coolant_IN_Pressure/1 -> En_OverRide_Batt_Coolant_IN_Pressure_port/1
  Val_OverRide_Batt_Coolant_IN_Pressure/1 -> Val_OverRide_Batt_Coolant_IN_Pressure_port/1
  En_OverRide_Batt_Coolant_IN_Temp/1 -> En_OverRide_Batt_Coolant_IN_Temp_port/1
  Val_OverRide_Batt_Coolant_IN_Temp/1 -> Val_OverRide_Batt_Coolant_IN_Temp_port/1
  En_OverRide_Batt_Coolant_OUT_Pressure/1 -> En_OverRide_Batt_Coolant_OUT_Pressure_port/1
  Val_OverRide_Batt_Coolant_OUT_Pressure/1 -> Val_OverRide_Batt_Coolant_OUT_Pressure_port/1
  En_OverRide_Batt_Coolant_OUT_Temp/1 -> En_OverRide_Batt_Coolant_OUT_Temp_port/1
  Val_OverRide_Batt_Coolant_OUT_Temp/1 -> Val_OverRide_Batt_Coolant_OUT_Temp_port/1
  En_OverRide_Batt_LVBackupBattVoltage/1 -> En_OverRide_Batt_LVBackupBattVoltage_port/1
  Val_OverRide_Batt_LVBackupBattVoltage/1 -> Val_OverRide_Batt_LVBackupBattVoltage_port/1
  En_OverRide_Batt_ThermalRequest/1 -> En_OverRide_Batt_ThermalRequest_port/1
  Val_OverRide_Batt_ThermalRequest/1 -> Val_OverRide_Batt_ThermalRequest_port/1
  En_OverRide_Batt_Current/1 -> En_OverRide_Batt_Current_port/1
  Val_OverRide_Batt_Current/1 -> Val_OverRide_Batt_Current_port/1
  En_OverRide_Batt_Voltage/1 -> En_OverRide_Batt_Voltage_port/1
  Val_OverRide_Batt_Voltage/1 -> Val_OverRide_Batt_Voltage_port/1
  En_OverRide_BMS_AliveCounter2/1 -> En_OverRide_BMS_AliveCounter2_port/1
  Val_OverRide_BMS_AliveCounter2/1 -> Val_OverRide_BMS_AliveCounter2_port/1
  En_OverRide_Batt_DischargePowerLim/1 -> En_OverRide_Batt_DischargePowerLim_port/1
  Val_OverRide_Batt_DischargePowerLim/1 -> Val_OverRide_Batt_DischargePowerLim_port/1
  En_OverRide_Batt_RegenPowerLim/1 -> En_OverRide_Batt_RegenPowerLim_port/1
  Val_OverRide_Batt_RegenPowerLim/1 -> Val_OverRide_Batt_RegenPowerLim_port/1
  En_OverRide_BMS_AliveCounter3/1 -> En_OverRide_BMS_AliveCounter3_port/1
  Val_OverRide_BMS_AliveCounter3/1 -> Val_OverRide_BMS_AliveCounter3_port/1
  En_OverRide_Batt_DischargePowerLim_2s/1 -> En_OverRide_Batt_DischargePowerLim_2s_port/1
  Val_OverRide_Batt_DischargePowerLim_2s/1 -> Val_OverRide_Batt_DischargePowerLim_2s_port/1
  En_OverRide_Batt_DischargePowerLim_5s/1 -> En_OverRide_Batt_DischargePowerLim_5s_port/1
  Val_OverRide_Batt_DischargePowerLim_5s/1 -> Val_OverRide_Batt_DischargePowerLim_5s_port/1
  En_OverRide_Batt_RegenPowerLim_2s/1 -> En_OverRide_Batt_RegenPowerLim_2s_port/1
  Val_OverRide_Batt_RegenPowerLim_2s/1 -> Val_OverRide_Batt_RegenPowerLim_2s_port/1
  En_OverRide_Batt_RegenPowerLim_5s/1 -> En_OverRide_Batt_RegenPowerLim_5s_port/1
  Val_OverRide_Batt_RegenPowerLim_5s/1 -> Val_OverRide_Batt_RegenPowerLim_5s_port/1
  En_OverRide_Batt_EnergyAvailable/1 -> En_OverRide_Batt_EnergyAvailable_port/1
  Val_OverRide_Batt_EnergyAvailable/1 -> Val_OverRide_Batt_EnergyAvailable_port/1
  En_OverRide_Batt_Isolation1Res_HighRange/1 -> En_OverRide_Batt_Isolation1Res_HighRange_port/1
  Val_OverRide_Batt_Isolation1Res_HighRange/1 -> Val_OverRide_Batt_Isolation1Res_HighRange_port/1
  En_OverRide_Batt_Isolation1Resistance/1 -> En_OverRide_Batt_Isolation1Resistance_port/1
  Val_OverRide_Batt_Isolation1Resistance/1 -> Val_OverRide_Batt_Isolation1Resistance_port/1
  En_OverRide_Batt_LVVoltage/1 -> En_OverRide_Batt_LVVoltage_port/1
  Val_OverRide_Batt_LVVoltage/1 -> Val_OverRide_Batt_LVVoltage_port/1
  En_OverRide_Batt_MaxCellTemperature/1 -> En_OverRide_Batt_MaxCellTemperature_port/1
  Val_OverRide_Batt_MaxCellTemperature/1 -> Val_OverRide_Batt_MaxCellTemperature_port/1
  En_OverRide_Batt_MaxCellVoltage/1 -> En_OverRide_Batt_MaxCellVoltage_port/1
  Val_OverRide_Batt_MaxCellVoltage/1 -> Val_OverRide_Batt_MaxCellVoltage_port/1
  En_OverRide_Batt_MinCellTemperature/1 -> En_OverRide_Batt_MinCellTemperature_port/1
  Val_OverRide_Batt_MinCellTemperature/1 -> Val_OverRide_Batt_MinCellTemperature_port/1
  En_OverRide_Batt_MinCellVoltage/1 -> En_OverRide_Batt_MinCellVoltage_port/1
  Val_OverRide_Batt_MinCellVoltage/1 -> Val_OverRide_Batt_MinCellVoltage_port/1
  En_OverRide_Batt_SerialNumber/1 -> En_OverRide_Batt_SerialNumber_port/1
  Val_OverRide_Batt_SerialNumber/1 -> Val_OverRide_Batt_SerialNumber_port/1
  En_OverRide_BMS_Calibration_info/1 -> En_OverRide_BMS_Calibration_info_port/1
  Val_OverRide_BMS_Calibration_info/1 -> Val_OverRide_BMS_Calibration_info_port/1
  En_OverRide_BMS_Software_info/1 -> En_OverRide_BMS_Software_info_port/1
  Val_OverRide_BMS_Software_info/1 -> Val_OverRide_BMS_Software_info_port/1
  En_OverRide_CIM_ChargePlugLockStatusHV/1 -> En_OverRide_CIM_ChargePlugLockStatusHV_port/1
  Val_OverRide_CIM_ChargePlugLockStatusHV/1 -> Val_OverRide_CIM_ChargePlugLockStatusHV_port/1
  En_OverRide_CIM_ChargeStatusHV/1 -> En_OverRide_CIM_ChargeStatusHV_port/1
  Val_OverRide_CIM_ChargeStatusHV/1 -> Val_OverRide_CIM_ChargeStatusHV_port/1
  En_OverRide_CIM_ChargingPlugTypeHV/1 -> En_OverRide_CIM_ChargingPlugTypeHV_port/1
  Val_OverRide_CIM_ChargingPlugTypeHV/1 -> Val_OverRide_CIM_ChargingPlugTypeHV_port/1
  En_OverRide_CIM_PlugPresentHV/1 -> En_OverRide_CIM_PlugPresentHV_port/1
  Val_OverRide_CIM_PlugPresentHV/1 -> Val_OverRide_CIM_PlugPresentHV_port/1
